simulink model "WSCC_Indian_400kV_Legacy"  (R2022a)
settings: Solver=FixedStepDiscrete  StartTime=0.0  StopTime=1  FixedStep=5e-7  RelTol=1e-3
PreLoadFcn:
  | tf=1e-3
  | to=20e-3
model workspace (MAT data in the model file):
  tf = 0.001
  to = 0.02
undefined symbols (not defined in the file or in its folder): D1, Delta
libraries: spsFourierLib x72, spsPowerPositiveSequenceLib x24, spsThreePhaseVIMeasurementLib x21, spsThreePhaseBreakerLib x12, spsDistributedParametersLineLib x12, spsLoadFlowBusLib x9, spsRMSLib x6, spsThreePhaseParallelRLCLoadLib x6, spsThreePhaseSeriesRLCLoadLib x3, spsThreePhaseSourceLib x3, spsThreePhaseTransformerTwoWindingsLib x3, spsThreePhaseFaultLib x1
(part 1 of 2)
settings Model: ParameterArgumentNames=tf,to  Creator=MARI  LastModifiedBy=Dell
settings SolverCC: AlgebraicLoopSolver=TrustRegion
settings DataIOCC: SignalLogging=off  DSMLogging=off  LoggingIntervals=[0, inf]
settings DebuggingCC: SFMachineParentedDataDiag=warning  ArithmeticOperatorsInVariantConditions=warning
settings SFSimCC: SimUseLocalCustomCode=off  CustomCodeUndefinedFunction=UseInterfaceOnly
settings RTWCC: RTWUseLocalCustomCode=off  DLArmComputeVersion=19.05

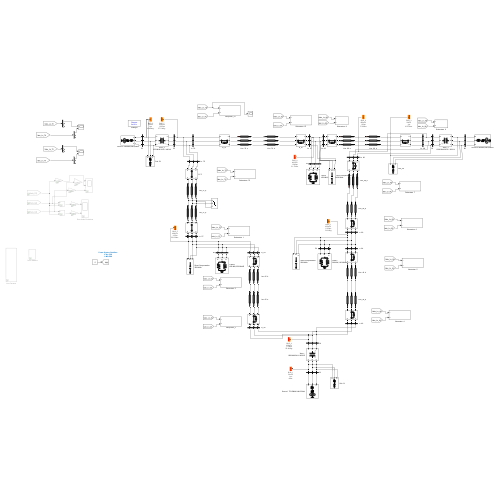
[thumbnail: Simulink's stored preview of the top-level diagram]
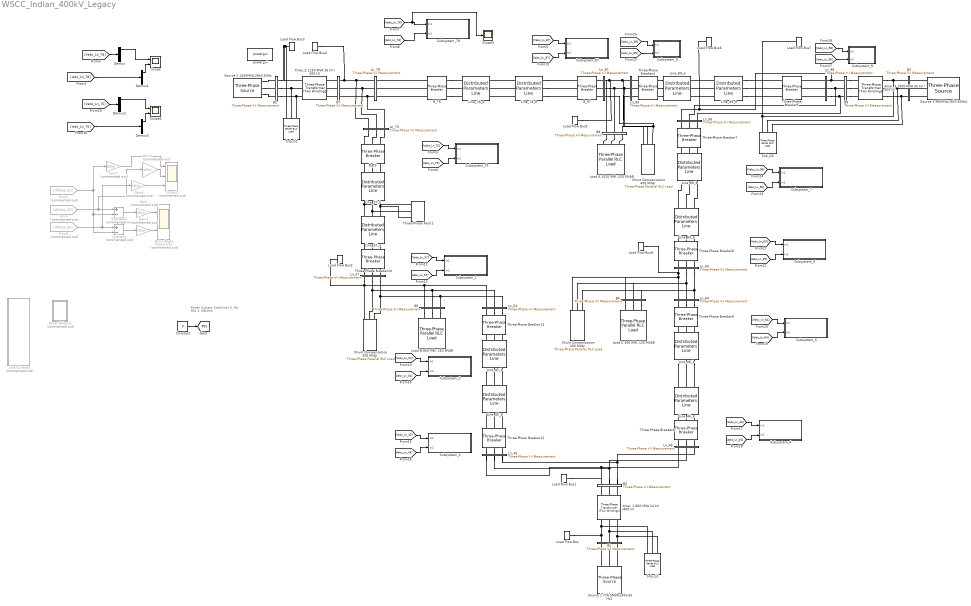
== system WSCC_Indian_400kV_Legacy ==
  note: Power System Stabilizer
      | 0: No PSS
      | 1: MB-PSS
  B1 : spsThreePhaseVIMeasurementLib/Three-Phase V-I Measurement  VoltageMeasurement=phase-to-ground  SetLabelV=on  LabelV=Vabc_G1  Vpu=off  VpuLL=off  CurrentMeasurement=yes  SetLabelI=on  LabelI=Iabc_G1  Ipu=off  Pbase=100e6  Vbase=500e3  OutputType=Complex  PhasorSimulation=off  PSBequivalent=0
  B2 : spsThreePhaseVIMeasurementLib/Three-Phase V-I Measurement  VoltageMeasurement=phase-to-ground  SetLabelV=on  LabelV=Vabc_G2  Vpu=off  VpuLL=off  CurrentMeasurement=yes  SetLabelI=on  LabelI=Iabc_G2  Ipu=off  Pbase=100e6  Vbase=500e3  OutputType=Complex  PhasorSimulation=off  PSBequivalent=0
  B3 : spsThreePhaseVIMeasurementLib/Three-Phase V-I Measurement  VoltageMeasurement=phase-to-ground  SetLabelV=on  LabelV=Vabc_G3  Vpu=off  VpuLL=off  CurrentMeasurement=yes  SetLabelI=on  LabelI=Iabc_G3  Ipu=off  Pbase=100e6  Vbase=500e3  OutputType=Complex  PhasorSimulation=off  PSBequivalent=0
  B4 : spsThreePhaseVIMeasurementLib/Three-Phase V-I Measurement  VoltageMeasurement=phase-to-ground  SetLabelV=on  LabelV=Vabc_X1  Vpu=off  VpuLL=off  CurrentMeasurement=yes  SetLabelI=on  LabelI=Iabc_X1  Ipu=off  Pbase=100e6  Vbase=500e3  OutputType=Complex  PhasorSimulation=off  PSBequivalent=0
  B5 : spsThreePhaseVIMeasurementLib/Three-Phase V-I Measurement  VoltageMeasurement=phase-to-ground  SetLabelV=on  LabelV=Vabc_Ld_B  Vpu=off  VpuLL=off  CurrentMeasurement=yes  SetLabelI=on  LabelI=Iabc_Ld_B  Ipu=off  Pbase=100e6  Vbase=500e3  OutputType=Complex  PhasorSimulation=off  PSBequivalent=0
  B6 : spsThreePhaseVIMeasurementLib/Three-Phase V-I Measurement  VoltageMeasurement=phase-to-ground  SetLabelV=on  LabelV=Vabc_Ld_C  Vpu=off  VpuLL=off  CurrentMeasurement=yes  SetLabelI=on  LabelI=Iabc_Ld_C  Ipu=off  Pbase=100e6  Vbase=500e3  OutputType=Complex  PhasorSimulation=off  PSBequivalent=0
  B7 : spsThreePhaseVIMeasurementLib/Three-Phase V-I Measurement  VoltageMeasurement=phase-to-ground  SetLabelV=on  LabelV=Vabc_X2  Vpu=off  VpuLL=off  CurrentMeasurement=yes  SetLabelI=on  LabelI=Iabc_X2  Ipu=off  Pbase=100e6  Vbase=500e3  OutputType=Complex  PhasorSimulation=off  PSBequivalent=0
  B8 : spsThreePhaseVIMeasurementLib/Three-Phase V-I Measurement  VoltageMeasurement=phase-to-ground  SetLabelV=on  LabelV=Vabc_Ld_A  Vpu=off  VpuLL=off  CurrentMeasurement=yes  SetLabelI=on  LabelI=Iabc_Ld_A  Ipu=off  Pbase=100e6  Vbase=500e3  OutputType=Complex  PhasorSimulation=off  PSBequivalent=0
  B9 : spsThreePhaseVIMeasurementLib/Three-Phase V-I Measurement  VoltageMeasurement=phase-to-ground  SetLabelV=on  LabelV=Vabc_X3  Vpu=off  VpuLL=off  CurrentMeasurement=yes  SetLabelI=on  LabelI=Iabc_X3  Ipu=off  Pbase=100e6  Vbase=500e3  OutputType=Complex  PhasorSimulation=off  PSBequivalent=0
  B_75 : spsThreePhaseBreakerLib/Three-Phase Breaker  InitialState=closed  SwitchA=on  SwitchB=on  SwitchC=on  SwitchTimes=[(0.5+(10/50)) ]  External=off  BreakerResistance=0.01  SnubberResistance=inf  SnubberCapacitance=inf  Measurements=None
  B_78 : spsThreePhaseBreakerLib/Three-Phase Breaker  InitialState=closed  SwitchA=on  SwitchB=on  SwitchC=on  SwitchTimes=[500 501]  External=off  BreakerResistance=0.01  SnubberResistance=10e6  SnubberCapacitance=inf  Measurements=None
  B_87 : spsThreePhaseBreakerLib/Three-Phase Breaker  InitialState=closed  SwitchA=on  SwitchB=on  SwitchC=on  SwitchTimes=[500 501]  External=off  BreakerResistance=0.01  SnubberResistance=10e6  SnubberCapacitance=inf  Measurements=None
  Constant : Constant  Value=0
  Demux{,1..3} (4 alike) : Demux  Outputs=3
  From : From  Commented=on  GotoTag=dtheta_G2
  From1 : From  Commented=on  GotoTag=dtheta_G1
  From2 : From  Commented=on  GotoTag=dtheta_G3
  Gain{,1..4} (5 alike) : Gain  Commented=on  Gain=180/pi
  Line Currents : Subsystem  Commented=on
  Line_45_a : spsDistributedParametersLineLib/Distributed Parameters Line  Phases=3  Length=75  Frequency=50  Resistance=[0.0298 0.1619]  Inductance=[1.0568e-03 3.9470e-03]  Capacitance=[11.0414e-09 7.1301e-09]  x1=[-0.0004 -0.000502991998355344 0 0;-0.00038 -0.000503285101497421 0 0;-0.00036 -0.000503558335805453 0 0;-0.00034 -0.000503811690492617 0 0;-0.00032 -0.000504045155556905 0 0;-0.0003 -0.000504258721781514 0 0;-0.00028 -0.000504452380735217 0 0;-0.00026 -0.000504626124772689 321740.825999906 -262623.935279686;-0.00024 -0.000504779947034814 323384.5791028 -260597.20737983;-0.00022 -0.000504913841448951 325015.565536233 -258560.19154844;-0.0002 -0.000505027802729179 326633.720911655 -256512.968203414;-0.00018 -0.000505121826376501 328238.981347062 -254455.618165624;-0.00016 -0.000505195908679025 329831.283469521 -252388.222655726;-0.00014 -0.000505250046712109 331410.564417669 -250310.863290956;-0.00012 -0.000505284238338474 332976.761844201 -248223.622081904;-0.0001 -0.000505298482208296 334529.813918322 -246126.581429279;-8e-05 -0.000505292777759249 336069.659328196 -244019.824120655;-6e-05 -0.000505267125216536 337596.237283364 -241903.433327204;-4e-05 -0.000505221525592876 339109.487517141 -239777.492600411;-2e-05 -0.000505155980688463 340609.350288999 -237642.085868774]  x2=[-0.0004 -0.000305148640405144 0 0;-0.00038 -0.000306750512833648 0 0;-0.00036 -0.000308340275277147 0 0;-0.00034 -0.000309917864974541 0 0;-0.00032 -0.00031148321964529 0 0;-0.0003 -0.000313036277491872 0 0;-0.00028 -0.000314576977202222 0 0;-0.00026 -0.000316105257952155 311271.717606713 -279950.706951068;-0.00024 -0.000317621059407763 313024.543961436 -277989.415950935;-0.00022 -0.0003191243217278 314765.012643147 -276017.150404654;-0.0002 -0.000320614985566043 316493.054941124 -274033.988173893;-0.00018 -0.000322092992073637 318208.602635214 -272040.0075505;-0.00016 -0.000323558282901415 319911.587998532 -270035.287253415;-0.00014 -0.000325010800202205 321601.943800133 -268019.906425565;-0.00012 -0.00032645048663311 323279.603307663 -265993.944630732;-0.0001 -0.000327877285357777 324944.500289998 -263957.48185042;-8e-05 -0.000329291140048632 326596.569019855 -261910.598480692;-6e-05 -0.000330691994889116 328235.744276391 -259853.375328999;-4e-05 -0.000332079794575877 329861.961347772 -257785.893610988;-2e-05 -0.000333454484320959 331475.156033733 -255708.234947298]  x3=[-0.0004 1.79056945115255e-06 0 0;-0.00038 1.80115317620371e-06 0 0;-0.00036 1.81166579481155e-06 0 0;-0.00034 1.82210689195587e-06 0 0;-0.00032 1.83247605544005e-06 0 0;-0.0003 1.84277287590726e-06 0 0;-0.00028 1.85299694685666e-06 0 0;-0.00026 1.86314786465944e-06 274.455148622571 -531.709356408434;-0.00024 1.87322522857474e-06 277.790537542582 -529.974419725581;-0.00022 1.88322864076549e-06 281.114959767823 -528.218560560099;-0.0002 1.89315770631411e-06 284.428284055799 -526.441848230301;-0.00018 1.90301203323809e-06 287.73037960214 -524.644352877748;-0.00016 1.91279123250548e-06 291.021116045767 -522.826145464478;-0.00014 1.92249491805023e-06 294.300363474041 -520.987297770207;-0.00012 1.93212270678745e-06 297.567992427888 -519.127882389493;-0.0001 1.94167421862854e-06 300.823873906911 -517.247972728872;-8e-05 1.95114907649615e-06 304.067879374486 -515.347643003957;-6e-05 1.96054690633912e-06 307.299880762831 -513.426968236514;-4e-05 1.96986733714723e-06 310.519750478065 -511.486024251492;-2e-05 1.97911000096581e-06 313.727361405245 -509.524887674037]  x4=[-0.0004 -2.83815574986041e-06 0 0;-0.00038 -2.85167951589665e-06 0 0;-0.00036 -2.86509070250846e-06 0 0;-0.00034 -2.87838878024516e-06 0 0;-0.00032 -2.89157322412141e-06 0 0;-0.0003 -2.90464351363793e-06 0 0;-0.00028 -2.91759913280208e-06 0 0;-0.00026 -2.9304395701482e-06 1690.23052973685 -1294.68064107459;-0.00024 -2.94316431875781e-06 1698.33183087633 -1284.03512342686;-0.00022 -2.95577287627961e-06 1706.36608478314 -1273.33891427108;-0.0002 -2.96826474494935e-06 1714.33297427868 -1262.59243587526;-0.00018 -2.98063943160945e-06 1722.23218484381 -1251.79611249199;-0.00016 -2.99289644772846e-06 1730.06340463121 -1240.95037034161;-0.00014 -3.00503530942037e-06 1737.82632447774 -1230.05563759546;-0.00012 -3.01705553746371e-06 1745.52063791662 -1219.11234435892;-0.0001 -3.02895665732046e-06 1753.14604118952 -1208.12092265449;-8e-05 -3.04073819915478e-06 1760.70223325858 -1197.08180640467;-6e-05 -3.05239969785157e-06 1768.18891581828 -1185.99543141486;-4e-05 -3.06394069303484e-06 1775.60579330721 -1174.86223535616;-2e-05 -3.07536072908586e-06 1782.95257291974 -1163.68265774811]  x5=0.000397871322084792  V1=[1.62e-10 4.153e+05 4.153e+05;314.2 314.2 314.2;-0.6943 0.8874 -0.6834]  V2=[8.471e-10 4.186e+05 4.186e+05;314.2 314.2 314.2;-0.039 0.8395 -0.7313]  I1=[7.601e-12 598 598;314.2 314.2 314.2;-1.312 0.4775 -1.093]  I2=[4.421e-12 2129 2129;314.2 314.2 314.2;2.105 0.9183 -0.6525]  nHarmo=1  Measurements=None  Decoupling=off  VsMag0=0  VrMag0=0  VsAngle0=0  VrAngle0=0  IsMag0=0  IrMag0=0  IsAngle0=0  IrAngle0=0
      settings: SourceProductBaseCode=PS
  Line_45_b : spsDistributedParametersLineLib/Distributed Parameters Line  Phases=3  Length=75  Frequency=50  Resistance=[0.0298 0.1619]  Inductance=[1.0568e-03 3.9470e-03]  Capacitance=[11.0414e-09 7.1301e-09]  x1=[-0.0004 -0.000305148627791813 0 0;-0.00038 -0.000306750500118396 0 0;-0.00036 -0.000308340262460476 0 0;-0.00034 -0.000309917852056956 0 0;-0.00032 -0.000311483206627302 0 0;-0.0003 -0.000313036264373994 0 0;-0.00028 -0.000314576963984974 0 0;-0.00026 -0.000316105244636057 311271.717606713 -279950.706951068;-0.00024 -0.00031762104599334 313024.543961436 -277989.415950935;-0.00022 -0.000319124308215583 314765.012643147 -276017.150404654;-0.0002 -0.000320614971956565 316493.054941124 -274033.988173893;-0.00018 -0.000322092978367435 318208.602635214 -272040.0075505;-0.00016 -0.00032355826909903 319911.587998532 -270035.287253415;-0.00014 -0.000325010786304183 321601.943800133 -268019.906425565;-0.00012 -0.000326450472639999 323279.603307663 -265993.944630732;-0.0001 -0.000327877271270129 324944.500289998 -263957.48185042;-8e-05 -0.000329291125867004 326596.569019855 -261910.598480692;-6e-05 -0.000330691980614067 328235.744276391 -259853.375328999;-4e-05 -0.000332079780207971 329861.961347772 -257785.893610988;-2e-05 -0.000333454469860763 331475.156033733 -255708.234947298]  x2=[-0.0004 -0.000103064623526066 0 0;-0.00038 -0.000105946361861863 0 0;-0.00036 -0.000108823917616703 0 0;-0.00034 -0.000111697177189612 0 0;-0.00032 -0.000114566027149221 0 0;-0.0003 -0.000117430354238247 0 0;-0.00028 -0.000120290045377961 0 0;-0.00026 -0.000123144987672653 298949.882553439 -295284.144230629;-0.00024 -0.000125995068414089 300799.294324294 -293399.970425258;-0.00022 -0.000128840175085963 302636.83105406 -291504.213691436;-0.0002 -0.000131680195368334 304462.420199933 -289596.948870392;-0.00018 -0.000134515017142064 306275.989690779 -287678.251257676;-0.00016 -0.000137344528493244 308077.467929982 -285748.196600185;-0.00014 -0.000140168617717611 309866.783798263 -283806.861093171;-0.00012 -0.000142987173324957 311643.866656497 -281854.321377236;-0.0001 -0.000145800084043534 313408.646348495 -279890.654535305;-8e-05 -0.000148607238824443 315161.053203777 -277915.938089583;-6e-05 -0.000151408526846019 316901.018040321 -275930.249998493;-4e-05 -0.000154203837518208 318628.472167293 -273933.668653602;-2e-05 -0.000156993060486931 320343.347387764 -271926.272876522]  x3=[-0.0004 2.02786013516334e-06 0 0;-0.00038 2.03713024797852e-06 0 0;-0.00036 2.04631993837963e-06 0 0;-0.00034 2.05542884357343e-06 0 0;-0.00032 2.06445660395595e-06 0 0;-0.0003 2.07340286312666e-06 0 0;-0.00028 2.08226726790257e-06 0 0;-0.00026 2.09104946833215e-06 311.165075108754 -505.329069968942;-0.00024 2.09974911770918e-06 314.333988267489 -503.364000256953;-0.00022 2.10836587258638e-06 317.490492058594 -501.37905859613;-0.0002 2.11689939278903e-06 320.634461868702 -499.374323348573;-0.00018 2.12534934142837e-06 323.765773579271 -497.349873657795;-0.00016 2.13371538491489e-06 326.884303571474 -495.305789445605;-0.00014 2.14199719297152e-06 329.989928731088 -493.242151408947;-0.00012 2.15019443864666e-06 333.082526453349 -491.159041016718;-0.0001 2.15830679832708e-06 336.161974647794 -489.056540506547;-8e-05 2.16633395175072e-06 339.228151743082 -486.934732881557;-6e-05 2.1742755820193e-06 342.28093669179 -484.793701907078;-4e-05 2.18213137561086e-06 345.320208975196 -482.633532107348;-2e-05 2.18990102239212e-06 348.345848608036 -480.454308762171]  x4=[-0.0004 -2.51020404096927e-06 0 0;-0.00038 -2.52564213893374e-06 0 0;-0.00036 -2.54098052887116e-06 0 0;-0.00034 -2.55621860524815e-06 0 0;-0.00032 -2.57135576649156e-06 0 0;-0.0003 -2.58639141501217e-06 0 0;-0.00028 -2.60132495722833e-06 0 0;-0.00026 -2.61615580358936e-06 1576.01556289566 -1423.10339701304;-0.00024 -2.63088336859883e-06 1584.92601720433 -1413.17297349099;-0.00022 -2.64550707083772e-06 1593.77390134767 -1403.18676031967;-0.0002 -2.66002633298727e-06 1602.55886602637 -1393.14515173771;-0.00018 -2.6744405818519e-06 1611.28056442505 -1383.0485441706;-0.00016 -2.68874924838173e-06 1619.93865222601 -1372.89733621512;-0.00014 -2.70295176769511e-06 1628.53278762276 -1362.69192862359;-0.00012 -2.71704757910089e-06 1637.06263133354 -1352.43272428801;-0.0001 -2.73103612612059e-06 1645.52784661474 -1342.12012822422;-8e-05 -2.7449168565103e-06 1653.92809927415 -1331.75454755584;-6e-05 -2.75868922228258e-06 1662.26305768418 -1321.33639149826;-4e-05 -2.77235267972799e-06 1670.53239279494 -1310.86607134243;-2e-05 -2.78590668943663e-06 1678.73577814725 -1300.34400043866]  x5=0.000397871322084792  V1=[8.377e-10 4.186e+05 4.186e+05;314.2 314.2 314.2;-0.02057 0.8395 -0.7313]  V2=[8.866e-10 4.202e+05 4.202e+05;314.2 314.2 314.2;-0.5299 0.7927 -0.7781]  I1=[5.663e-12 593.1 593.1;314.2 314.2 314.2;-2.774 0.5529 -1.018]  I2=[8.582e-12 2124 2124;314.2 314.2 314.2;-0.07241 0.8375 -0.7333]  nHarmo=1  Measurements=None  Decoupling=off  VsMag0=0  VrMag0=0  VsAngle0=0  VrAngle0=0  IsMag0=0  IrMag0=0  IsAngle0=0  IrAngle0=0
      settings: SourceProductBaseCode=PS
  Line_46_a : spsDistributedParametersLineLib/Distributed Parameters Line  Phases=3  Length=90  Frequency=50  Resistance=[0.0298 0.1619]  Inductance=[1.0568e-03 3.9470e-03]  Capacitance=[11.0414e-09 7.1301e-09]  x1=[-0.00048 -0.000501780155719701 302839.15593119 -284220.468288801;-0.00046 -0.000502153472113537 304618.976263006 -282312.076006295;-0.00044 -0.000502506964348118 306386.77075923 -280392.538526423;-0.00042 -0.000502840618468176 308142.469630363 -278461.931629239;-0.0004 -0.000503154421301618 309886.003564419 -276520.331531798;-0.00038 -0.000503448360460045 311617.303729664 -274567.814885147;-0.00036 -0.000503722424339243 313336.301777333 -272604.458771299;-0.00034 -0.000503976602119639 315042.929844324 -270630.340700193;-0.00032 -0.00050421088376673 316737.120555886 -268645.538606629;-0.0003 -0.000504425260031477 318418.807028269 -266650.130847196;-0.00028 -0.000504619722450672 320087.92287137 -264644.196197175;-0.00026 -0.000504794263347272 321744.402191355 -262627.813847432;-0.00024 -0.000504948875830701 323388.179593256 -260601.063401288;-0.00022 -0.000505083553797124 325019.190183556 -258564.024871383;-0.0002 -0.000505198291929684 326637.36957275 -256516.778676508;-0.00018 -0.000505293085698717 328242.653877885 -254459.405638437;-0.00016 -0.000505367931361927 329834.979725087 -252391.986978737;-0.00014 -0.000505422825964535 331414.284252057 -250314.604315555;-0.00012 -0.000505457767339397 332980.505110557 -248227.339660401;-0.0001 -0.000505472754107086 334533.58046887 -246130.275414912;-8e-05 -0.000505467785675951 336073.449014239 -244023.494367591;-6e-05 -0.000505442862242137 337600.04995529 -241907.079690548;-4e-05 -0.000505397984789579 339113.323024433 -239781.11493621;-2e-05 -0.000505333155089961 340613.208480238 -237645.684034025]  x2=[-0.00048 -0.000411589322638186 301824.904517896 -295099.84373655;-0.00046 -0.000412724558984348 303673.101552408 -293197.609392173;-0.00044 -0.000413843501671618 305509.310092842 -291283.800108212;-0.00042 -0.000414946106526057 307333.45764883 -289358.491438581;-0.0004 -0.000416032330018711 309145.472206149 -287421.759391168;-0.00038 -0.000417102129267337 310945.282229567 -285473.68042484;-0.00036 -0.000418155462038093 312732.816665666 -283514.331446418;-0.00034 -0.000419192286747205 314508.004945647 -281543.789807644;-0.00032 -0.000420212562462608 316270.776988118 -279562.13330213;-0.0003 -0.000421216248905564 318021.063201855 -277569.440162279;-0.00028 -0.000422203306452252 319758.794488556 -275565.789056206;-0.00026 -0.000423173696135328 321483.902245565 -273551.259084625;-0.00024 -0.00042412737964547 323196.318368583 -271525.92977773;-0.00022 -0.000425064319332886 324895.975254352 -269489.881092055;-0.0002 -0.000425984478208802 326582.805803329 -267443.193407314;-0.00018 -0.000426887819946921 328256.743422332 -265385.947523234;-0.00016 -0.000427774308884856 329917.72202717 -263318.22465636;-0.00014 -0.000428643910025544 331565.676045253 -261240.106436848;-0.00012 -0.00042949658903862 333200.540418176 -259151.67490525;-0.0001 -0.000430332312261777 334822.250604295 -257053.012509265;-8e-05 -0.000431151046702093 336430.742581267 -254944.202100491;-6e-05 -0.000431952760037334 338025.952848584 -252825.326931153;-4e-05 -0.00043273742061723 339607.818430075 -250696.470650814;-2e-05 -0.000433504997464725 341176.276876397 -248557.717303074]  x3=[-0.00048 5.03743589015423e-07 565.121573651507 -958.528765308815;-0.00046 5.07008815739957e-07 571.132992855913 -954.959104569544;-0.00044 5.10254026624583e-07 577.121864707697 -951.351743679977;-0.00042 5.13479093553934e-07 583.087952776453 -947.706825052544;-0.0004 5.16683889207888e-07 589.031021531241 -944.024492582392;-0.00038 5.198682870666e-07 594.950836349881 -940.304891641702;-0.00036 5.23032161415496e-07 600.84716352822 -936.54816907395;-0.00034 5.26175387350234e-07 606.719770289359 -932.75447318811;-0.00032 5.29297840781636e-07 612.568424792837 -928.9239537528;-0.0003 5.32399398440587e-07 618.39289614379 -925.056761990368;-0.00028 5.35479937882902e-07 624.192954402061 -921.153050570924;-0.00026 5.38539337494157e-07 629.968370591282 -917.21297360631;-0.00024 5.41577476494495e-07 635.718916707911 -913.236686644018;-0.00022 5.4459423494339e-07 641.444365730233 -909.224346661049;-0.0002 5.47589493744385e-07 647.144491627325 -905.176112057716;-0.00018 5.50563134649789e-07 652.819069367976 -901.092142651388;-0.00016 5.53515040265353e-07 658.467874929574 -896.972599670185;-0.00014 5.56445094054897e-07 664.090685306947 -892.817645746611;-0.00012 5.59353180344914e-07 669.687278521169 -888.627444911131;-0.0001 5.62239184329137e-07 675.257433628324 -884.402162585699;-8e-05 5.6510299207307e-07 680.800930728226 -880.141965577228;-6e-05 5.67944490518488e-07 686.317550973099 -875.847022071;-4e-05 5.70763567487897e-07 691.807076576225 -871.517501624032;-2e-05 5.73560111688965e-07 697.269290820531 -867.153575158376]  x4=[-0.00048 -1.68914033558431e-06 1286.57292882659 -995.934322856657;-0.00046 -1.694977924365e-06 1292.80513169933 -987.830941038064;-0.00044 -1.70074859831951e-06 1298.98629683911 -979.688561345357;-0.00042 -1.7064521296315e-06 1305.11618022411 -971.507505225743;-0.0004 -1.71208829313533e-06 1311.19453985704 -963.28809565331;-0.00038 -1.71765686632491e-06 1317.22113577465 -955.030657116274;-0.00036 -1.7231576293625e-06 1323.19573005727 -946.735515604169;-0.00034 -1.72859036508741e-06 1329.11808683814 -938.40299859498;-0.00032 -1.73395485902453e-06 1334.98797231275 -930.033435042209;-0.0003 -1.73925089939281e-06 1340.80515474808 -921.627155361894;-0.00028 -1.74447827711367e-06 1346.56940449173 -913.184491419565;-0.00026 -1.74963678581917e-06 1352.28049398099 -904.705776517137;-0.00024 -1.75472622186022e-06 1357.93819775182 -896.191345379756;-0.00022 -1.7597463843146e-06 1363.54229244776 -887.641534142585;-0.0002 -1.7646970749949e-06 1369.09255682876 -879.056680337532;-0.00018 -1.76957809845633e-06 1374.58877177988 -870.437122879925;-0.00016 -1.77438926200443e-06 1380.03072031996 -861.783202055134;-0.00014 -1.77913037570271e-06 1385.41818761019 -853.095259505135;-0.00012 -1.78380125238012e-06 1390.75096096259 -844.373638215024;-0.0001 -1.78840170763844e-06 1396.0288298484 -835.618682499475;-8e-05 -1.79293155985957e-06 1401.25158590639 -826.83073798915;-6e-05 -1.79739063021271e-06 1406.41902295109 -818.01015161705;-4e-05 -1.8017787426614e-06 1411.53093698095 -809.157271604822;-2e-05 -1.80609572397047e-06 1416.58712618634 -800.272447449009]  x5=0.00047744558650175  V1=[2.78e-10 4.153e+05 4.153e+05;314.2 314.2 314.2;2.169 0.8713 -0.6995]  V2=[5.247e-10 4.221e+05 4.221e+05;314.2 314.2 314.2;2.009 0.8508 -0.72]  I1=[2.389e-12 1113 1113;314.2 314.2 314.2;0.1121 0.5869 -0.9839]  I2=[3.387e-12 1627 1627;314.2 314.2 314.2;-2.917 0.9662 -0.6046]  nHarmo=1  Measurements=None  Decoupling=off  VsMag0=0  VrMag0=0  VsAngle0=0  VrAngle0=0  IsMag0=0  IrMag0=0  IsAngle0=0  IrAngle0=0
      settings: SourceProductBaseCode=PS
  Line_46_b : spsDistributedParametersLineLib/Distributed Parameters Line  Phases=3  Length=30  Frequency=50  Resistance=[0.0298 0.1619]  Inductance=[1.0568e-03 3.9470e-03]  Capacitance=[11.0414e-09 7.1301e-09]  x1=[-0.00016 -0.000427774308702069 0 0;-0.00014 -0.000428643909865589 0 0;-0.00012 -0.000429496588901504 333200.540418176 -259151.67490525;-0.0001 -0.000430332312147506 334822.250604295 -257053.012509265;-8e-05 -0.00043115104661067 336430.742581267 -254944.202100491;-6e-05 -0.000431952759968763 338025.952848584 -252825.326931153;-4e-05 -0.000432737420571515 339607.818430075 -250696.470650814;-2e-05 -0.000433504997441867 341176.276876397 -248557.717303074]  x2=[-0.00016 -0.000399750126995155 0 0;-0.00014 -0.000400886003436956 0 0;-0.00012 -0.000402006053585768 332630.691588008 -262198.669447582;-0.0001 -0.000403110233223929 334271.557727847 -260103.527348785;-8e-05 -0.000404198498760318 335899.227398951 -257998.116808096;-6e-05 -0.000405270807232074 337513.636343708 -255882.520943518;-4e-05 -0.000406327116306296 339114.720828019 -253756.823275156;-2e-05 -0.00040736738428171 340702.417643809 -251621.107721911]  x3=[-0.00016 6.4357650210188e-07 0 0;-0.00014 6.4602632630302e-07 0 0;-0.00012 6.48450646490972e-07 753.040289841409 -823.678614845093;-0.0001 6.50849366957726e-07 758.200716781565 -818.930895583143;-8e-05 6.53222393005905e-07 763.33121125567 -814.150846331669;-6e-05 6.55569630952504e-07 768.431570720586 -809.338655798831;-4e-05 6.57890988132588e-07 773.501593822857 -804.494513961673;-2e-05 6.6018637290295e-07 778.54108040665 -799.618612058618]  x4=[-0.00016 -1.7395987457411e-06 0 0;-0.00014 -1.74490522315752e-06 0 0;-0.00012 -1.75014281470349e-06 1367.39693584155 -892.4465672657;-0.0001 -1.75531131360786e-06 1372.97731485002 -883.837399334052;-8e-05 -1.76041051582714e-06 1378.50349106502 -875.193339015251;-6e-05 -1.76544022005356e-06 1383.97524632256 -866.514727561996;-4e-05 -1.77040022772301e-06 1389.39236460713 -857.801907591008;-2e-05 -1.77529034302289e-06 1394.75463206016 -849.0552230695]  x5=0.000159148528833917  V1=[5.267e-10 4.221e+05 4.221e+05;314.2 314.2 314.2;2.115 0.9152 -0.6556]  V2=[4.511e-10 4.235e+05 4.235e+05;314.2 314.2 314.2;1.521 0.9087 -0.6621]  I1=[7.622e-12 1116 1116;314.2 314.2 314.2;-1.047 0.7461 -0.8247]  I2=[9.859e-12 1633 1633;314.2 314.2 314.2;1.521 0.998 -0.5728]  nHarmo=1  Measurements=None  Decoupling=off  VsMag0=0  VrMag0=0  VsAngle0=0  VrAngle0=0  IsMag0=0  IrMag0=0  IsAngle0=0  IrAngle0=0
      settings: SourceProductBaseCode=PS
  Line_57_a : spsDistributedParametersLineLib/Distributed Parameters Line  Phases=3  Length=30  Frequency=50  Resistance=[0.0298 0.1619]  Inductance=[1.0568e-03 3.9470e-03]  Capacitance=[11.0414e-09 7.1301e-09]  x1=[-0.00016 -0.000137305305694705 0 0;-0.00014 -0.00014012931010315 0 0;-0.00012 -0.000142947782446373 311649.17374747 -281855.555955426;-0.0001 -0.00014576061145591 313413.961091743 -279891.85574391;-8e-05 -0.000148567686086089 315166.375389483 -277917.10588118;-6e-05 -0.00015136889551841 316906.347458374 -275931.38432698;-4e-05 -0.000154164129165921 318633.808607298 -273934.769474197;-2e-05 -0.000156953276677584 320348.690639046 -271927.340145767]  x2=[-0.00016 -0.000142819253464008 0 0;-0.00014 -0.000145971796518761 0 0;-0.00012 -0.000149118576856932 318234.770516593 -270572.457865407;-0.0001 -0.000152259470249021 319928.534537009 -268567.602119856;-8e-05 -0.000155394352697934 321609.668326686 -266552.143785234;-6e-05 -0.00015852310044388 323278.105517342 -264526.162428386;-4e-05 -0.000161645589969256 324933.780241933 -262489.738031587;-2e-05 -0.000164761698003521 326576.627137255 -260442.950989384]  x3=[-0.00016 1.19106734480895e-06 0 0;-0.00014 1.18519076420232e-06 0 0;-0.00012 1.17926739429368e-06 2171.66168617045 -1479.63388710976;-0.0001 1.17329746892755e-06 2180.91557213176 -1465.95981740172;-8e-05 1.16728122378635e-06 2190.08335928061 -1452.22787411021;-6e-05 1.16121889638114e-06 2199.16468568846 -1438.43859934884;-4e-05 1.15511072604223e-06 2208.15919284009 -1424.59253749457;-2e-05 1.14895695390972e-06 2217.06652564776 -1410.69023516622]  x4=[-0.00016 -1.53383949725334e-06 0 0;-0.00014 -1.53601602750111e-06 0 0;-0.00012 -1.53813191846619e-06 -168.781227025331 -334.859258343707;-0.0001 -1.54018708661683e-06 -166.673926497094 -335.913125247926;-8e-05 -1.54218145081851e-06 -164.56004596763 -336.953730877135;-6e-05 -1.54411493233716e-06 -162.439668889323 -337.981034150007;-4e-05 -1.54598745484222e-06 -160.31287897103 -338.994994510367;-2e-05 -1.54779894440972e-06 -158.179760174774 -339.995571928796]  x5=0.000159148528833917  V1=[8.847e-10 4.202e+05 4.202e+05;314.2 314.2 314.2;0.04885 0.841 -0.7298]  V2=[4.139e-10 4.177e+05 4.177e+05;314.2 314.2 314.2;-0.2267 0.8716 -0.6992]  I1=[1.496e-11 2628 2628;314.2 314.2 314.2;1.536 0.9781 -0.5927]  I2=[1.402e-11 375 375;314.2 314.2 314.2;-1.159 -0.4607 -2.031]  nHarmo=1  Measurements=None  Decoupling=off  VsMag0=0  VrMag0=0  VsAngle0=0  VrAngle0=0  IsMag0=0  IrMag0=0  IsAngle0=0  IrAngle0=0
      settings: SourceProductBaseCode=PS
  Line_57_b : spsDistributedParametersLineLib/Distributed Parameters Line  Phases=3  Length=90  Frequency=50  Resistance=[0.0298 0.1619]  Inductance=[1.0568e-03 3.9470e-03]  Capacitance=[11.0414e-09 7.1301e-09]  x1=[-0.00048 -9.16970319348276e-05 285665.838008779 -304758.680171657;-0.00046 -9.49247126624822e-05 287575.041868576 -302957.78491149;-0.00044 -9.8148645925018e-05 289472.892758129 -301144.929396722;-0.00042 -0.00010136870444707 291359.315753532 -299320.185195783;-0.0004 -0.000104584761106242 293234.236382036 -297483.624346452;-0.00038 -0.000107796688938123 295097.580624985 -295635.319353005;-0.00036 -0.000111004361141302 296949.274920739 -293775.343183358;-0.00034 -0.000114207651082373 298789.246167578 -291903.769266187;-0.00032 -0.000117406432300934 300617.421726588 -290020.671488024;-0.0003 -0.00012060057851458 302433.729424527 -288126.124190346;-0.00028 -0.000123789963623888 304238.097556678 -286220.202166635;-0.00026 -0.000126974461717394 306030.454889676 -284302.980659431;-0.00024 -0.000130153947076566 307810.730664324 -282374.535357355;-0.00022 -0.000133328294180767 309578.854598381 -280434.942392125;-0.0002 -0.000136497377712209 311334.756889342 -278484.278335552;-0.00018 -0.000139661072560899 313078.368217192 -276522.620196511;-0.00016 -0.000142819253829583 314809.619747141 -274550.045417908;-0.00014 -0.000145971796838672 316528.443132343 -272566.631873616;-0.00012 -0.000149118577131164 318234.770516593 -270572.457865407;-0.0001 -0.000152259470477564 319928.534537009 -268567.602119856;-8e-05 -0.000155394352880779 321609.668326686 -266552.143785234;-6e-05 -0.00015852310058102 323278.105517342 -264526.162428386;-4e-05 -0.000161645590060686 324933.780241933 -262489.738031587;-2e-05 -0.000164761698049237 326576.627137255 -260442.950989384]  x2=[-0.00048 -9.21193518598346e-05 307474.163519976 -271342.512180013;-0.00046 -9.62856591401417e-05 309172.978307394 -269405.251677202;-0.00044 -0.000100448165227493 310859.587475018 -267457.355516351;-0.00042 -0.000104606705793277 312533.924438405 -265498.900597064;-0.0004 -0.000108761116665431 314195.923097598 -263529.964235789;-0.00038 -0.000112911233834927 315845.517839738 -261550.624162761;-0.00036 -0.000117056893462248 317482.643541647 -259560.958518937;-0.00034 -0.000121197931883847 319107.235572407 -257561.045852911;-0.00032 -0.00012533418561862 320719.229795905 -255550.96511781;-0.0003 -0.000129465491374351 322318.562573371 -253530.795668179;-0.00028 -0.000133591686054164 323905.170765883 -251500.617256849;-0.00026 -0.000137712606762956 325478.991736869 -249460.510031788;-0.00024 -0.000141828090813835 327039.96335457 -247410.554532936;-0.00022 -0.000145937975734538 328588.023994499 -245350.831689026;-0.0002 -0.000150042099273844 330123.112541875 -243281.422814388;-0.00018 -0.000154140299407984 331645.168394028 -241202.409605743;-0.00016 -0.000158232414347034 333154.131462801 -239113.87413897;-0.00014 -0.000162318282541303 334649.942176914 -237015.898865876;-0.00012 -0.000166397742687711 336132.541484324 -234908.56661093;-0.0001 -0.000170470633736155 337601.870854546 -232791.960568002;-8e-05 -0.000174536794895873 339057.872280974 -230666.164297075;-6e-05 -0.000178596065641783 340500.488283165 -228531.261720945;-4e-05 -0.000182648285720826 341929.661909108 -226387.337121911;-2e-05 -0.000186693295158294 343345.336737476 -224234.475138444]  x3=[-0.00048 1.23785488124962e-06 2040.99402128711 -1646.0438750609;-0.00046 1.2324041301442e-06 2051.29606442935 -1633.18752431424;-0.00044 1.22690472583395e-06 2061.51712591535 -1620.26669812058;-0.00042 1.22135688542591e-06 2071.65680223509 -1607.28190657202;-0.0004 1.21576082793934e-06 2081.71469309153 -1594.23366228589;-0.00038 1.21011677429699e-06 2091.69040141636 -1581.12248038455;-0.00036 1.20442494731645e-06 2101.58353338568 -1567.94887847499;-0.00034 1.19868557170129e-06 2111.39369843559 -1554.71337662847;-0.00032 1.19289887403224e-06 2121.12050927757 -1541.41649735993;-0.0003 1.18706508275822e-06 2130.76358191379 -1528.05876560741;-0.00028 1.18118442818731e-06 2140.32253565225 -1514.64070871128;-0.00026 1.17525714247768e-06 2149.79699312181 -1501.16285639345;-0.00024 1.16928345962843e-06 2159.18658028713 -1487.62574073645;-0.00022 1.16326361547033e-06 2168.49092646338 -1474.02989616243;-0.0002 1.15719784765652e-06 2177.7096643309 -1460.37585941205;-0.00018 1.15108639565312e-06 2186.84242994972 -1446.66416952331;-0.00016 1.1449295007298e-06 2195.88886277387 -1432.89536781024;-0.00014 1.13872740595022e-06 2204.84860566568 -1419.06999784155;-0.00012 1.13248035616247e-06 2213.72130490985 -1405.18860541919;-0.0001 1.12618859798938e-06 2222.5066102274 -1391.25173855676;-8e-05 1.11985237981878e-06 2231.20417478951 -1377.25994745789;-6e-05 1.11347195179372e-06 2239.81365523124 -1363.21378449455;-4e-05 1.10704756580257e-06 2248.33471166504 -1349.11380418519;-2e-05 1.10057947546909e-06 2256.76700769418 -1334.96056317289]  x4=[-0.00048 -1.36356553672137e-06 -225.806870609764 -296.28896755923;-0.00046 -1.36802539695598e-06 -223.940787135922 -297.701896136061;-0.00044 -1.37243124989035e-06 -222.065862863252 -299.10307195178;-0.00042 -1.37678292158896e-06 -220.182171810554 -300.492439690365;-0.0004 -1.38108024025525e-06 -218.289788342725 -301.869944501957;-0.00038 -1.38532303623845e-06 -216.388787167824 -303.235532005023;-0.00036 -1.38951114204023e-06 -214.479243334123 -304.589148288509;-0.00034 -1.39364439232134e-06 -212.561232227142 -305.93073991396;-0.00032 -1.39772262390815e-06 -210.634829566676 -307.260253917637;-0.0003 -1.40174567579905e-06 -208.700111403803 -308.577637812603;-0.00028 -1.40571338917084e-06 -206.757154117884 -309.882839590798;-0.00026 -1.409625607385e-06 -204.806034413545 -311.17580772509;-0.00024 -1.41348217599384e-06 -202.846829317652 -312.456491171311;-0.00022 -1.41728294274664e-06 -200.879616176267 -313.724839370272;-0.0002 -1.42102775759564e-06 -198.904472651596 -314.980802249758;-0.00018 -1.42471647270196e-06 -196.921476718923 -316.224330226504;-0.00016 -1.42834894244144e-06 -194.930706663534 -317.455374208156;-0.00014 -1.4319250234104e-06 -192.93224107762 -318.673885595205;-0.00012 -1.43544457443128e-06 -190.926158857181 -319.879816282907;-0.0001 -1.43890745655824e-06 -188.912539198909 -321.073118663185;-8e-05 -1.44231353308262e-06 -186.891461597059 -322.253745626503;-6e-05 -1.44566266953835e-06 -184.863005840315 -323.421650563731;-4e-05 -1.44895473370726e-06 -182.827252008636 -324.576787367981;-2e-05 -1.45218959562428e-06 -180.784280470098 -325.71911043643]  x5=0.00047744558650175  V1=[4.309e-10 4.177e+05 4.177e+05;314.2 314.2 314.2;-0.354 0.8072 -0.7636]  V2=[3.73e-10 4.101e+05 4.101e+05;314.2 314.2 314.2;-0.5088 0.9019 -0.6689]  I1=[1.704e-12 2622 2622;314.2 314.2 314.2;-1.588 0.9462 -0.6246]  I2=[3.147e-12 372.5 372.5;314.2 314.2 314.2;-0.7702 -0.5974 -2.168]  nHarmo=1  Measurements=None  Decoupling=off  VsMag0=0  VrMag0=0  VsAngle0=0  VrAngle0=0  IsMag0=0  IrMag0=0  IsAngle0=0  IrAngle0=0
      settings: SourceProductBaseCode=PS
  Line_69_a : spsDistributedParametersLineLib/Distributed Parameters Line  Phases=3  Length=70  Frequency=50  Resistance=[0.0298 0.1619]  Inductance=[1.0568e-03 3.9470e-03]  Capacitance=[11.0414e-09 7.1301e-09]  x1=[-0.00038 -0.000386210445846985 310131.617493116 -288465.740037434;-0.00036 -0.000387517233677351 311937.967531581 -286511.444371006;-0.00034 -0.000388808722990867 313732.002793211 -284545.837723341;-0.00032 -0.000390084862801746 315513.652452566 -282568.997693223;-0.0003 -0.000391345602730174 317282.846173168 -280581.002322911;-0.00028 -0.000392590893004298 319039.514110279 -278581.930095059;-0.00026 -0.000393820684462189 320783.586913655 -276571.859929616;-0.00024 -0.000395034928553786 322514.99573029 -274550.87118071;-0.00022 -0.000396233577342812 324233.672207128 -272519.043633515;-0.0002 -0.000397416583508665 325939.548493763 -270476.457501106;-0.00018 -0.000398583900348288 327632.557245122 -268423.193421284;-0.00016 -0.000399735481778009 329312.631624118 -266359.3324534;-0.00014 -0.000400871282335367 330979.705304291 -264284.956075151;-0.00012 -0.0004019912571809 332633.712472426 -262200.146179365;-0.0001 -0.000403095362099919 334274.587831153 -260104.985070766;-8e-05 -0.000404183553504251 335902.266601523 -257999.555462727;-6e-05 -0.000405255788433965 337516.684525563 -255883.940474005;-4e-05 -0.00040631202455906 339117.77786882 -253758.223625456;-2e-05 -0.000407352220181143 340705.483422869 -251622.488836743]  x2=[-0.00038 -0.000329528474463061 316167.909351575 -274630.341663344;-0.00036 -0.000330896720690628 317887.210439041 -272638.392204937;-0.00034 -0.000332251903682248 319593.961883749 -270635.679449638;-0.00032 -0.000333593969937617 321288.096306073 -268622.282461116;-0.0003 -0.000334922866474258 322969.546824489 -266598.280724838;-0.00028 -0.00033623854082961 324638.247058209 -264563.754144927;-0.00026 -0.000337540941063102 326294.131129805 -262518.783041007;-0.00024 -0.000338830015758204 327937.133667809 -260463.448145037;-0.00022 -0.000340105714024454 329567.189809294 -258397.83059812;-0.0002 -0.000341367985499468 331184.235202434 -256322.011947298;-0.00018 -0.000342616780350931 332788.206009047 -254236.074142338;-0.00016 -0.000343852049278559 334379.038907112 -252140.099532493;-0.00014 -0.00034507374351605 335956.671093269 -250034.170863251;-0.00012 -0.000346281814833009 337521.040285301 -247918.371273071;-0.0001 -0.000347476215536847 339072.084724592 -245792.784290097;-8e-05 -0.00034865689847467 340609.743178561 -243657.493828864;-6e-05 -0.000349823817035138 342133.954943088 -241512.584186983;-4e-05 -0.000350976925150304 343644.6598449 -239358.140041814;-2e-05 -0.000352116177297434 345141.798243956 -237194.246447123]  x3=[-0.00038 -3.05530268384323e-07 1574.64888181013 -1169.47388647692;-0.00036 -3.03535352930101e-07 1581.96577236795 -1159.55705644633;-0.00034 -3.01528454419881e-07 1589.22020962585 -1149.59444908862;-0.00032 -2.9950965208258e-07 1596.41190719105 -1139.58645771049;-0.0003 -2.97479025617057e-07 1603.54058114764 -1129.53347741029;-0.00028 -2.95436655188968e-07 1610.6059500678 -1119.43590506247;-0.00026 -2.93382621427601e-07 1617.60773502284 -1109.2941393019;-0.00024 -2.91317005422692e-07 1624.5456595943 -1099.10858050813;-0.00022 -2.89239888721224e-07 1631.41944988478 -1088.87963078957;-0.0002 -2.87151353324206e-07 1638.22883452882 -1078.60769396766;-0.00018 -2.85051481683442e-07 1644.97354470357 -1068.29317556085;-0.00016 -2.82940356698266e-07 1651.65331413941 -1057.93648276869;-0.00014 -2.8081806171228e-07 1658.2678791305 -1047.53802445566;-0.00012 -2.78684680510055e-07 1664.81697854513 -1037.0982111351;-0.0001 -2.76540297313828e-07 1671.30035383608 -1026.61745495296;-8e-05 -2.74384996780176e-07 1677.71774905077 -1016.09616967155;-6e-05 -2.72218863996673e-07 1684.06891084145 -1005.5347706532;-4e-05 -2.70041984478533e-07 1690.35358847511 -994.933674843854;-2e-05 -2.67854444165232e-07 1696.57153384346 -984.293300756623]  x4=[-0.00038 -6.12185239320934e-07 371.3787512776 -717.272178732514;-0.00036 -6.18085617328539e-07 375.878144937533 -714.924594240005;-0.00034 -6.23961594374304e-07 380.36269957191 -712.548785748662;-0.00032 -6.29812938484716e-07 384.832238138194 -710.144847051336;-0.0003 -6.3563941865873e-07 389.286584186654 -707.712873051412;-0.00028 -6.41440804876884e-07 393.725561867336 -705.252959759058;-0.00026 -6.47216868110384e-07 398.148995937001 -702.76520428744;-0.00024 -6.52967380330143e-07 402.556711766047 -700.249704848882;-0.00022 -6.58692114515787e-07 406.948535345401 -697.706560750997;-0.0002 -6.64390844664611e-07 411.324293293386 -695.135872392759;-0.00018 -6.70063345800507e-07 415.683812862572 -692.537741260542;-0.00016 -6.75709393982843e-07 420.026921946591 -689.912269924114;-0.00014 -6.81328766315305e-07 424.353449086932 -687.259562032589;-0.00012 -6.86921240954693e-07 428.663223479714 -684.579722310331;-0.0001 -6.92486597119687e-07 432.956074982421 -681.872856552825;-8e-05 -6.98024615099554e-07 437.231834120627 -679.139071622496;-6e-05 -7.03535076262825e-07 441.490332094683 -676.378475444491;-4e-05 -7.09017763065931e-07 445.731400786381 -673.591177002421;-2e-05 -7.14472459061784e-07 449.95487276559 -670.777286334056]  x5=0.000371346567279139  V1=[7.818e-10 4.235e+05 4.235e+05;314.2 314.2 314.2;1.708 0.8658 -0.705]  V2=[9.391e-10 4.188e+05 4.188e+05;314.2 314.2 314.2;1.235 0.8998 -0.671]  I1=[4.724e-12 1961 1961;314.2 314.2 314.2;-0.8175 0.9762 -0.5946]  I2=[5.7e-12 807.8 807.8;314.2 314.2 314.2;1.598 0.522 -1.049]  nHarmo=1  Measurements=None  Decoupling=off  VsMag0=0  VrMag0=0  VsAngle0=0  VrAngle0=0  IsMag0=0  IrMag0=0  IsAngle0=0  IrAngle0=0
      settings: SourceProductBaseCode=PS
  Line_69_b : spsDistributedParametersLineLib/Distributed Parameters Line  Phases=3  Length=70  Frequency=50  Resistance=[0.0298 0.1619]  Inductance=[1.0568e-03 3.9470e-03]  Capacitance=[11.0414e-09 7.1301e-09]  x1=[-0.00038 -0.000329528461531173 316167.909351575 -274630.341663344;-0.00036 -0.000330896707668672 317887.210439041 -272638.392204937;-0.00034 -0.000332251890570739 319593.961883749 -270635.679449638;-0.00032 -0.000333593956737073 321288.096306073 -268622.282461116;-0.0003 -0.000334922853185199 322969.546824489 -266598.280724838;-0.00028 -0.000336238527452561 324638.247058209 -264563.754144927;-0.00026 -0.000337540927598591 326294.131129805 -262518.783041007;-0.00024 -0.000338830002206763 327937.133667809 -260463.448145037;-0.00022 -0.000340105700386617 329567.189809294 -258397.83059812;-0.0002 -0.000341367971775775 331184.235202434 -256322.011947298;-0.00018 -0.000342616766541922 332788.206009047 -254236.074142338;-0.00016 -0.00034385203538478 334379.038907112 -252140.099532493;-0.00014 -0.000345073729538051 335956.671093269 -250034.170863251;-0.00012 -0.000346281800771339 337521.040285301 -247918.371273071;-0.0001 -0.000347476201392063 339072.084724592 -245792.784290097;-8e-05 -0.000348656884247331 340609.743178561 -243657.493828864;-6e-05 -0.000349823802725804 342133.954943088 -241512.584186983;-4e-05 -0.00035097691075954 343644.6598449 -239358.140041814;-2e-05 -0.000352116162825808 345141.798243956 -237194.246447123]  x2=[-0.00038 -0.000268754608279637 320559.859976877 -259085.927766452;-0.00036 -0.000270162036121011 322181.406580677 -257066.689883258;-0.00034 -0.00027155879842779 323790.234014208 -255037.303447317;-0.00032 -0.000272944840058191 325386.278763717 -252997.848575329;-0.0003 -0.000274320106293663 326969.477820092 -250948.405781481;-0.00028 -0.00027568454284105 328539.768681344 -248889.055974265;-0.00026 -0.000277038095834732 330097.089355078 -246819.880453286;-0.00024 -0.000278380711838757 331641.378360941 -244740.96090605;-0.00022 -0.000279712337848942 333172.574733048 -242652.379404741;-0.0002 -0.000281032921294973 334690.618022387 -240554.21840298;-0.00018 -0.000282342410042477 336195.448299209 -238446.560732572;-0.00016 -0.00028364075239508 337687.00615539 -236329.489600232;-0.00014 -0.000284927897096449 339165.232706782 -234203.088584303;-0.00012 -0.000286203793332316 340630.069595529 -232067.441631457;-0.0001 -0.000287468390732481 342081.458992382 -229922.633053378;-8e-05 -0.000288721639372804 343519.343598971 -227768.747523437;-6e-05 -0.000289963489777176 344943.666650073 -225605.870073347;-4e-05 -0.000291193892919469 346354.371915855 -223434.086089805;-2e-05 -0.000292412800225473 347751.403704087 -221253.481311125]  x3=[-0.00038 -2.63555567121397e-07 1662.23209254417 -1049.16655312505;-0.00036 -2.61291402545705e-07 1668.79134598867 -1038.70179993513;-0.00034 -2.59016922632844e-07 1675.28471840826 -1028.19604057668;-0.00032 -2.56732217175385e-07 1681.71195345571 -1017.64968979911;-0.0003 -2.54437376369588e-07 1688.07279739479 -1007.06316395429;-0.00028 -2.52132490811839e-07 1694.36699911027 -996.436880980115;-0.00026 -2.49817651495072e-07 1700.59431011785 -985.771260384055;-0.00024 -2.4749294980518e-07 1706.75448457395 -975.066723226546;-0.00022 -2.45158477517407e-07 1712.84727928542 -964.323692104386;-0.0002 -2.42814326792719e-07 1718.87245371918 -953.542591134048;-0.00018 -2.40460590174174e-07 1724.82977001165 -942.723845934938;-0.00016 -2.38097360583263e-07 1730.71899297818 -931.867883612593;-0.00014 -2.35724731316245e-07 1736.53989012233 -920.975132741816;-0.00012 -2.3334279604046e-07 1742.29223164505 -910.046023349761;-0.0001 -2.30951648790634e-07 1747.97579045375 -899.080986898952;-8e-05 -2.28551383965166e-07 1753.59034217125 -888.080456270253;-6e-05 -2.26142096322402e-07 1759.13566514467 -877.044865745778;-4e-05 -2.23723880976893e-07 1764.61154045416 -865.974650991745;-2e-05 -2.21296833395639e-07 1770.01775192153 -854.870249041277]  x4=[-0.00038 -4.96869478284107e-07 320.889568163653 -744.355774623379;-0.00036 -5.03115356453991e-07 325.560128569359 -742.32488633027;-0.00034 -5.09341372491074e-07 330.217836418638 -740.264692321711;-0.00032 -5.15547280602902e-07 334.862507833159 -738.175273930636;-0.0003 -5.21732835790851e-07 339.493959449247 -736.056713643705;-0.00028 -5.27897793859793e-07 344.112008425122 -733.90909509805;-0.00026 -5.34041911427738e-07 348.716472448119 -731.732503077975;-0.00024 -5.40164945935447e-07 353.307169741882 -729.527023511604;-0.00022 -5.46266655656001e-07 357.883919073543 -727.292743467496;-0.0002 -5.52346799704348e-07 362.446539760874 -725.0297511512;-0.00018 -5.58405138046812e-07 366.994851679423 -722.738135901779;-0.00016 -5.64441431510568e-07 371.528675269623 -720.417988188278;-0.00014 -5.70455441793087e-07 376.047831543883 -718.069399606156;-0.00012 -5.7644693147154e-07 380.55214209365 -715.69246287367;-0.0001 -5.82415664012174e-07 385.041429096458 -713.287271828212;-8e-05 -5.88361403779647e-07 389.515515322941 -710.853921422605;-6e-05 -5.94283916046336e-07 393.974224143836 -708.392507721357;-4e-05 -6.00182967001597e-07 398.417379536954 -705.903127896866;-2e-05 -6.06058323760998e-07 402.844806094128 -703.385880225586]  x5=0.000371346567279139  V1=[9.514e-10 4.188e+05 4.188e+05;314.2 314.2 314.2;1.248 0.8998 -0.671]  V2=[3.385e-10 4.122e+05 4.122e+05;314.2 314.2 314.2;1.899 0.9353 -0.6355]  I1=[9.51e-12 1966 1966;314.2 314.2 314.2;2.181 1.052 -0.5188]  I2=[1.088e-11 810.7 810.7;314.2 314.2 314.2;-0.4113 0.4513 -1.119]  nHarmo=1  Measurements=None  Decoupling=off  VsMag0=0  VrMag0=0  VsAngle0=0  VrAngle0=0  IsMag0=0  IrMag0=0  IsAngle0=0  IrAngle0=0
      settings: SourceProductBaseCode=PS
  Line_78_a : spsDistributedParametersLineLib/Distributed Parameters Line  Phases=3  Length=100  Frequency=50  Resistance=[0.0298 0.1619]  Inductance=[1.0568e-03 3.9470e-03]  Capacitance=[11.0414e-09 7.1301e-09]  x1=[-0.00054 -7.86116219991208e-05 302306.480951241 -277089.945200239;-0.00052 -8.27932942288857e-05 304041.509693409 -275185.040541629;-0.0005 -8.69716979211592e-05 305764.535397377 -273269.272048811;-0.00048 -9.11466681197183e-05 307475.49004104 -271342.715353045;-0.00046 -9.5318040003888e-05 309174.306078839 -269405.446511489;-0.00044 -9.94856488950491e-05 310860.916444425 -267457.542004202;-0.00042 -0.000103649330263138 312535.254553309 -265499.078731116;-0.0004 -0.000107808919733145 314197.254305489 -263530.13400901;-0.00038 -0.000111964253091599 315846.850088061 -261550.785568449;-0.00036 -0.000116115166293055 317483.976777808 -259561.11155072;-0.00034 -0.000120261495466566 319108.569743772 -257561.190504747;-0.00032 -0.000124403076922157 320720.564849803 -255551.101383989;-0.0003 -0.000128539747157283 322319.898457096 -253530.923543321;-0.00028 -0.000132671342863287 323906.507426698 -251500.736735906;-0.00026 -0.000136797700931844 325480.329122003 -249460.621110043;-0.00024 -0.000140918658461404 327041.301411226 -247410.657206004;-0.00022 -0.000145034052763618 328589.362669854 -245350.925952853;-0.0002 -0.000149143721369768 330124.451783079 -243281.508665254;-0.00018 -0.000153247502037174 331646.508148211 -241202.487040257;-0.00016 -0.0001573452327556 333155.471677071 -239113.943154076;-0.00014 -0.000161436751753656 334651.282798363 -237015.959458849;-0.00012 -0.000165521897505176 336133.882460024 -234908.618779378;-0.0001 -0.000169600508735601 337603.21213156 -232792.004309866;-8e-05 -0.000173672424428345 339059.21380635 -230666.199610628;-6e-05 -0.000177737483831147 340501.830003941 -228531.288604793;-4e-05 -0.000181795526462422 341931.003772316 -226387.355574991;-2e-05 -0.000185846392117596 343346.678690142 -224234.485160029]  x2=[-0.00054 1.48220438794773e-05 278378.632660918 -309253.440627953;-0.00052 1.17895679991099e-05 280316.221591206 -307498.243205379;-0.0005 8.75662668678494e-06 282242.744117044 -305730.906278685;-0.00048 5.72333967783213e-06 284158.124182621 -303951.499619306;-0.00046 2.68982672122875e-06 286062.286172011 -302160.09347517;-0.00044 -3.43792425127842e-07 287955.154912161 -300356.758567925;-0.00042 -3.37739799914818e-06 289836.655675854 -298541.566090144;-0.0004 -6.41087023927853e-06 291706.714184659 -296714.58770252;-0.00038 -9.44408938922899e-06 293565.256611871 -294875.89553103;-0.00036 -1.24769357027013e-05 295412.209585416 -293025.562164092;-0.00034 -1.55092894481159e-05 297247.500190753 -291163.660649701;-0.00032 -1.85410309133393e-05 299071.055973752 -289290.264492539;-0.0003 -2.15720404104096e-05 300882.804943553 -287405.447651079;-0.00028 -2.46021982802617e-05 302682.675575409 -285509.284534663;-0.00026 -2.76313848974514e-05 304470.596813508 -283601.850000564;-0.00024 -3.06594806748779e-05 306246.498073783 -281683.219351031;-0.00022 -3.36863660685047e-05 308010.309246691 -279753.468330316;-0.0002 -3.67119215820795e-05 309761.960699989 -277812.673121687;-0.00018 -3.97360277718511e-05 311501.383281476 -275860.910344414;-0.00016 -4.27585652512853e-05 313228.508321726 -273898.257050751;-0.00014 -4.57794146957777e-05 314943.267636801 -271924.790722888;-0.00012 -4.87984568473648e-05 316645.593530939 -269940.589269897;-0.0001 -5.1815572519432e-05 318335.418799229 -267945.731024654;-8e-05 -5.48306426014185e-05 320012.676730262 -265940.294740747;-6e-05 -5.78435480635203e-05 321677.301108767 -263924.359589366;-4e-05 -6.08541699613885e-05 323329.226218224 -261898.00515618;-2e-05 -6.38623894408257e-05 324968.386843458 -259861.311438191]  x3=[-0.00054 -1.37818042793668e-06 -99.8584639562027 -314.331095974709;-0.00052 -1.37793540670088e-06 -97.8815053079144 -314.952316438569;-0.0005 -1.37763598693462e-06 -95.9006824653965 -315.56110312426;-0.00048 -1.37728218045849e-06 -93.9160736281432 -316.157431997927;-0.00046 -1.37687400124017e-06 -91.9277571451131 -316.741279517527;-0.00044 -1.37641146539386e-06 -89.9358115116364 -317.31262263376;-0.00042 -1.37589459117969e-06 -87.940315366316 -317.871438790977;-0.0004 -1.37532339900296e-06 -85.941347487923 -318.417705928074;-0.00038 -1.37469791141338e-06 -83.9389867922862 -318.951402479359;-0.00036 -1.37401815310412e-06 -81.9333123291775 -319.472507375407;-0.00034 -1.37328415091086e-06 -79.9244032791903 -319.981000043888;-0.00032 -1.37249593381077e-06 -77.9123389506141 -320.476860410383;-0.0003 -1.3716535329213e-06 -75.8971987763035 -320.960068899172;-0.00028 -1.37075698149899e-06 -73.879062310542 -321.430606434014;-0.00026 -1.36980631493817e-06 -71.8580092259017 -321.888454438891;-0.00024 -1.36880157076952e-06 -69.8341193100977 -322.333594838747;-0.00022 -1.36774278865862e-06 -67.8074724628386 -322.766010060203;-0.0002 -1.36663001040437e-06 -65.7781486926716 -323.185683032246;-0.00018 -1.36546327993736e-06 -63.7462281138245 -323.592597186905;-0.00016 -1.36424264331811e-06 -61.7117909430425 -323.986736459907;-0.00014 -1.36296814873525e-06 -59.6749174964215 -324.368085291307;-0.00012 -1.36163984650366e-06 -57.6356881862376 -324.736628626107;-0.0001 -1.36025778906242e-06 -55.5941835177722 -325.092351914847;-8e-05 -1.35882203097281e-06 -53.5504840861341 -325.435241114181;-6e-05 -1.35733262891609e-06 -51.5046705730773 -325.76528268743;-4e-05 -1.35578964169131e-06 -49.4568237438164 -326.082463605118;-2e-05 -1.35419313021296e-06 -47.4070244438378 -326.386771345485]  x4=[-0.00054 1.42135215849248e-06 1862.00304861866 -1667.59919523511;-0.00052 1.41152115450041e-06 1872.44406007242 -1655.86704506055;-0.0005 1.40163442607007e-06 1882.81115064083 -1644.06952409035;-0.00048 1.39169236351258e-06 1893.10391104891 -1632.20709807044;-0.00046 1.38169535932353e-06 1903.32193495608 -1620.28023530908;-0.00044 1.37164380816754e-06 1913.46481897227 -1608.2894066584;-0.00042 1.36153810686263e-06 1923.53216267379 -1596.23508549577;-0.0004 1.35137865436459e-06 1933.52356861914 -1584.11774770516;-0.00038 1.34116585175121e-06 1943.43864236472 -1571.93787165832;-0.00036 1.33090010220644e-06 1953.27699248041 -1559.69593819589;-0.00034 1.3205818110045e-06 1963.03823056497 -1547.39243060845;-0.00032 1.31021138549386e-06 1972.72197126145 -1535.02783461741;-0.0003 1.29978923508117e-06 1982.32783227235 -1522.60263835585;-0.00028 1.28931577121507e-06 1991.85543437472 -1510.11733234923;-0.00026 1.27879140736998e-06 2001.30440143514 -1497.57240949607;-0.00024 1.26821655902978e-06 2010.67436042458 -1484.96836504844;-0.00022 1.25759164367135e-06 2019.96494143309 -1472.30569659243;-0.0002 1.24691708074818e-06 2029.17577768445 -1459.58490402851;-0.00018 1.23619329167372e-06 2038.30650555061 -1446.80648955179;-0.00016 1.22542069980481e-06 2047.35676456607 -1433.97095763219;-0.00014 1.21459973042493e-06 2056.3261974421 -1421.07881499454;-0.00012 1.20373081072742e-06 2065.21445008085 -1408.13057059854;-0.0001 1.19281436979862e-06 2074.02117158933 -1395.12673561873;-8e-05 1.18185083860092e-06 2082.74601429324 -1382.06782342423;-6e-05 1.17084064995577e-06 2091.38863375075 -1368.95434955854;-4e-05 1.15978423852656e-06 2099.94868876602 -1355.78683171916;-2e-05 1.14868204080148e-06 2108.42584140275 -1342.56578973714]  x5=0.000530495096113056  V1=[8.92e-10 4.101e+05 4.101e+05;314.2 314.2 314.2;-0.7547 0.8912 -0.6796]  V2=[4.527e-10 4.161e+05 4.161e+05;314.2 314.2 314.2;-0.9521 0.7952 -0.7756]  I1=[5.472e-12 329.9 329.9;314.2 314.2 314.2;0.6215 -0.2451 -1.816]  I2=[4.185e-12 2499 2499;314.2 314.2 314.2;-1.63 0.9027 -0.6681]  nHarmo=1  Measurements=None  Decoupling=off  VsMag0=0  VrMag0=0  VsAngle0=0  VrAngle0=0  IsMag0=0  IrMag0=0  IsAngle0=0  IrAngle0=0
      settings: SourceProductBaseCode=PS
  Line_78_b : spsDistributedParametersLineLib/Distributed Parameters Line  Phases=3  Length=10  Frequency=50  Resistance=[0.0298 0.1619]  Inductance=[1.0568e-03 3.9470e-03]  Capacitance=[11.0414e-09 7.1301e-09]  x1=[-6e-05 -5.78435478578096e-05 0 0;-4e-05 -6.08541698242436e-05 323329.226218224 -261898.00515618;-2e-05 -6.38623893722518e-05 324968.386843458 -259861.311438191]  x2=[-6e-05 -4.58192365546322e-05 0 0;-4e-05 -4.87198961278785e-05 321274.698353668 -265270.987804589;-2e-05 -5.16186323230476e-05 322935.09246916 -263247.136401205]  x3=[-6e-05 -1.33717889238232e-06 0 0;-4e-05 -1.334073695538e-06 -22.6247847025794 -328.35354104521;-2e-05 -1.33091583174847e-06 -20.5612455358813 -328.489214392254]  x4=[-6e-05 1.20862508947825e-06 0 0;-4e-05 1.19758032147816e-06 2095.55384429237 -1385.57459717307;-2e-05 1.18648827505756e-06 2104.21824449844 -1372.38058064693]  x5=5.30495096113055e-05  V1=[4.527e-10 4.161e+05 4.161e+05;314.2 314.2 314.2;-0.8021 0.8918 -0.679]  V2=[3.459e-10 4.166e+05 4.166e+05;314.2 314.2 314.2;-1.332 0.8824 -0.6884]  I1=[2.305e-11 329.2 329.2;314.2 314.2 314.2;1.554 -0.06674 -1.638]  I2=[1.894e-11 2512 2512;314.2 314.2 314.2;-2.04 0.9884 -0.5824]  nHarmo=1  Measurements=None  Decoupling=off  VsMag0=0  VrMag0=0  VsAngle0=0  VrAngle0=0  IsMag0=0  IrMag0=0  IsAngle0=0  IrAngle0=0
      settings: SourceProductBaseCode=PS
  Line_89_a : spsDistributedParametersLineLib/Distributed Parameters Line  Phases=3  Length=100  Frequency=50  Resistance=[0.0298 0.1619]  Inductance=[1.0568e-03 3.9470e-03]  Capacitance=[11.0414e-09 7.1301e-09]  x1=[-0.00054 2.40426038328311e-05 275822.474002518 -312264.756805445;-0.00052 2.11301884881824e-05 277779.033922328 -310525.560654946;-0.0005 1.82169389598729e-05 279724.627601512 -308774.105487018;-0.00048 1.53029702580057e-05 281659.178231364 -307010.460446111;-0.00046 1.23883974210755e-05 283582.609439137 -305234.695157911;-0.00044 9.47333551142755e-06 285494.845291061 -303446.879726593;-0.00042 6.55789961071451e-06 287395.810295337 -301647.084732047;-0.0004 3.64220481535376e-06 289285.429405124 -299835.381227098;-0.00038 7.26366231983364e-07 291163.628021494 -298011.840734699;-0.00036 -2.18950102708214e-06 293030.331996382 -296176.535245106;-0.00034 -5.1052818483961e-06 294885.467635511 -294329.537213037;-0.00032 -8.02086112192435e-06 296728.961701302 -292470.919554811;-0.0003 -1.09361237455894e-05 298560.741415767 -290600.755645472;-0.00028 -1.38509546298146e-05 300380.734463378 -288719.119315888;-0.00026 -1.67652387020677e-05 302188.868993927 -286826.08484984;-0.00024 -1.96788609114035e-05 303985.073625359 -284921.726981087;-0.00022 -2.25917062330062e-05 305769.277446589 -283006.120890417;-0.0002 -2.55036596727299e-05 307541.410020307 -281079.342202678;-0.00018 -2.8414606271639e-05 309301.401385753 -279141.466983794;-0.00016 -3.13244311105462e-05 311049.18206148 -277192.57173776;-0.00014 -3.42330193145491e-05 312784.683048101 -275232.733403624;-0.00012 -3.71402560575657e-05 314507.835831009 -273262.029352446;-0.0001 -4.00460265668676e-05 316218.572383082 -271280.53738425;-8e-05 -4.29502161276103e-05 317916.82516737 -269288.335724944;-6e-05 -4.58527100873629e-05 319602.527139761 -267285.50302324;-4e-05 -4.87533938606337e-05 321275.611751628 -265272.118347542;-2e-05 -5.1652152933394e-05 322936.012952455 -263248.26118283]  x2=[-0.00054 -0.000231569722429994 304441.989310742 -278441.264238236;-0.00052 -0.000233188054019842 306185.466433075 -276522.915199255;-0.0005 -0.000234797179744598 307916.855877466 -274593.649509064;-0.00048 -0.000236397036078735 309636.089291625 -272653.543331771;-0.00046 -0.000237987559862664 311343.098803161 -270702.673259444;-0.00044 -0.00023956868830523 313037.817022261 -268741.116309094;-0.00042 -0.000241140358986188 314720.177044352 -266768.949919631;-0.0004 -0.000242702509858673 316390.11245274 -264786.251948807;-0.00038 -0.000244255079251641 318047.557321235 -262793.100670142;-0.00036 -0.000245798005872313 319692.446216751 -260789.574769837;-0.00034 -0.000247331228808586 321324.714201893 -258775.753343663;-0.00032 -0.000248854687531445 322944.296837513 -256751.715893842;-0.0003 -0.000250368321897347 324551.130185264 -254717.542325908;-0.00028 -0.0002518720721506 326145.150810115 -252673.312945548;-0.00026 -0.000253365878925719 327726.295782863 -250619.108455439;-0.00024 -0.000254849683249769 329294.50268261 -248555.009952057;-0.00022 -0.000256323426544697 330849.709599234 -246481.098922477;-0.0002 -0.000257787050629642 332391.855135828 -244397.457241154;-0.00018 -0.00025924049772323 333920.878411127 -242304.167166695;-0.00016 -0.000260683710445858 335436.719061911 -240201.311338607;-0.00014 -0.00026211663182196 336939.317245386 -238088.972774039;-0.00012 -0.000263539205282253 338428.613641549 -235967.234864498;-0.0001 -0.000264951374665973 339904.549455528 -233836.181372566;-8e-05 -0.000266353084223091 341367.066419904 -231695.896428585;-6e-05 -0.000267744278616513 342816.106797012 -229546.46452734;-4e-05 -0.000269124902924267 344251.613381218 -227387.970524722;-2e-05 -0.000270494902641669 345673.529501182 -225220.499634378]  x3=[-0.00054 -1.79504755453719e-06 1915.2535545649 -1812.17451505855;-0.00052 -1.81018420594905e-06 1926.60190244914 -1800.10493046174;-0.0005 -1.825249394388e-06 1937.87419138914 -1787.96428080455;-0.00048 -1.84024252510619e-06 1949.06997637423 -1775.75304537904;-0.00046 -1.85516300620048e-06 1960.188815414 -1763.47170626387;-0.00044 -1.87001024863584e-06 1971.23026955572 -1751.12074830529;-0.00042 -1.88478366626855e-06 1982.19390290168 -1738.70065909796;-0.0004 -1.89948267586938e-06 1993.07928262642 -1726.21192896575;-0.00038 -1.91410669714661e-06 2003.88597899377 -1713.65505094232;-0.00036 -1.92865515276891e-06 2014.61356537388 -1701.03052075174;-0.00034 -1.94312746838816e-06 2025.26161826 -1688.33883678882;-0.00032 -1.95752307266213e-06 2035.82971728523 -1675.58050009953;-0.0003 -1.97184139727701e-06 2046.31744523912 -1662.75601436115;-0.00028 -1.98608187696985e-06 2056.72438808414 -1649.86588586241;-0.00026 -2.00024394955091e-06 2067.05013497198 -1636.91062348353;-0.00024 -2.01432705592581e-06 2077.29427825985 -1623.89073867607;-0.00022 -2.02833064011762e-06 2087.45641352652 -1610.80674544279;-0.0002 -2.04225414928881e-06 2097.53613958828 -1597.65916031734;-0.00018 -2.0560970337631e-06 2107.5330585148 -1584.44850234388;-0.00016 -2.06985874704709e-06 2117.44677564485 -1571.17529305655;-0.00014 -2.08353874585191e-06 2127.27689960185 -1557.84005645894;-0.00012 -2.09713649011464e-06 2137.02304230933 -1544.44331900335;-0.0001 -2.11065144301961e-06 2146.68481900627 -1530.98560957003;-8e-05 -2.12408307101962e-06 2156.26184826226 -1517.46745944632;-6e-05 -2.137430843857e-06 2165.7537519926 -1503.88940230562;-4e-05 -2.15069423458453e-06 2175.16015547318 -1490.2519741864;-2e-05 -2.16387271958627e-06 2184.48068735529 -1476.55571347095]  x4=[-0.00054 1.60079146061387e-06 -155.21259206971 -183.683013449754;-0.00052 1.60979092552815e-06 -154.055421487093 -184.654610784829;-0.0005 1.6187268386531e-06 -152.892169060222 -185.618918272049;-0.00048 1.62759884721416e-06 -151.72288071231 -186.575897842207;-0.00046 1.63640660095963e-06 -150.547602604858 -187.525511715386;-0.00044 1.64514975217447e-06 -149.366381135834 -188.467722402459;-0.00042 1.65382795569404e-06 -148.179262937839 -189.402492706559;-0.0004 1.66244086891772e-06 -146.986294876267 -190.329785724556;-0.00038 1.67098815182246e-06 -145.787524047454 -191.24956484851;-0.00036 1.67946946697615e-06 -144.58299777682 -192.161793767115;-0.00034 1.687884479551e-06 -143.372763616999 -193.066436467136;-0.00032 1.69623285733672e-06 -142.156869345965 -193.963457234828;-0.0003 1.70451427075364e-06 -140.93536296514 -194.852820657347;-0.00028 1.71272839286575e-06 -139.708292697505 -195.734491624148;-0.00026 1.72087489939358e-06 -138.475706985693 -196.60843532837;-0.00024 1.72895346872698e-06 -137.237654490078 -197.474617268214;-0.00022 1.73696378193788e-06 -135.994184086853 -198.333003248298;-0.0002 1.74490552279283e-06 -134.745344866098 -199.183559381015;-0.00018 1.7527783777655e-06 -133.49118612985 -200.026252087864;-0.00016 1.76058203604904e-06 -132.231757390146 -200.86104810078;-0.00014 1.76831618956841e-06 -130.967108367078 -201.687914463447;-0.00012 1.77598053299245e-06 -129.697288986823 -202.506818532596;-0.0001 1.78357476374602e-06 -128.422349379677 -203.317727979296;-8e-05 1.79109858202188e-06 -127.142339878071 -204.120610790232;-6e-05 1.79855169079258e-06 -125.857311014589 -204.915435268963;-4e-05 1.80593379582213e-06 -124.567313519971 -205.702170037182;-2e-05 1.81324460567769e-06 -123.272398321108 -206.480784035947]  x5=0.000530495096113056  V1=[5.499e-10 4.166e+05 4.166e+05;314.2 314.2 314.2;-1.286 0.7858 -0.785]  V2=[5.945e-10 4.126e+05 4.126e+05;314.2 314.2 314.2;-0.5426 0.8923 -0.6785]  I1=[4.251e-12 2637 2637;314.2 314.2 314.2;-0.8207 0.8753 -0.6955]  I2=[3.147e-12 240.5 240.5;314.2 314.2 314.2;2.253 -0.6397 -2.211]  nHarmo=1  Measurements=None  Decoupling=off  VsMag0=0  VrMag0=0  VsAngle0=0  VrAngle0=0  IsMag0=0  IrMag0=0  IsAngle0=0  IrAngle0=0
      settings: SourceProductBaseCode=PS
  Line_89_b : spsDistributedParametersLineLib/Distributed Parameters Line  Phases=3  Length=10  Frequency=50  Resistance=[0.0298 0.1619]  Inductance=[1.0568e-03 3.9470e-03]  Capacitance=[11.0414e-09 7.1301e-09]  x1=[-6e-05 -0.000267744278616513 0 0;-4e-05 -0.000269124902924267 344251.613381218 -227387.970524722;-2e-05 -0.000270494902641669 345673.529501182 -225220.499634378]  x2=[-6e-05 -0.000289688472317203 0 0;-4e-05 -0.000290914043084836 346349.120271208 -223429.067650337;-2e-05 -0.000292128129064172 347746.12063153 -221248.495967559]  x3=[-6e-05 -2.53305858885099e-06 0 0;-4e-05 -2.54420970704731e-06 2346.56677919426 -1260.74061470193;-2e-05 -2.55526038420077e-06 2354.44187474426 -1245.97191184872]  x4=[-6e-05 1.78972865861669e-06 0 0;-4e-05 1.79734318268201e-06 -123.74462031454 -207.368426480706;-2e-05 1.80488675071601e-06 -122.439252025644 -208.141838489235]  x5=5.30495096113055e-05  V1=[5.916e-10 4.126e+05 4.126e+05;314.2 314.2 314.2;-0.4212 0.9888 -0.582]  V2=[6.139e-10 4.122e+05 4.122e+05;314.2 314.2 314.2;-0.1116 0.9997 -0.5711]  I1=[1.499e-11 2664 2664;314.2 314.2 314.2;1.83 1.08 -0.4912]  I2=[2.162e-11 241.5 241.5;314.2 314.2 314.2;2.618 -0.5367 -2.107]  nHarmo=1  Measurements=None  Decoupling=off  VsMag0=0  VrMag0=0  VsAngle0=0  VrAngle0=0  IsMag0=0  IrMag0=0  IsAngle0=0  IrAngle0=0
      settings: SourceProductBaseCode=PS
  Ln_45 : spsThreePhaseVIMeasurementLib/Three-Phase V-I Measurement  VoltageMeasurement=phase-to-ground  SetLabelV=on  LabelV=Vabc_Ln_45  Vpu=off  VpuLL=off  CurrentMeasurement=yes  SetLabelI=on  LabelI=Iabc_Ln_45  Ipu=off  Pbase=100e6  Vbase=500e3  OutputType=Complex  PhasorSimulation=off  PSBequivalent=0
  Ln_46 : spsThreePhaseVIMeasurementLib/Three-Phase V-I Measurement  VoltageMeasurement=phase-to-ground  SetLabelV=on  LabelV=Vabc_Ln_46  Vpu=off  VpuLL=off  CurrentMeasurement=yes  SetLabelI=on  LabelI=Iabc_Ln_46  Ipu=off  Pbase=100e6  Vbase=500e3  OutputType=Complex  PhasorSimulation=off  PSBequivalent=0
  Ln_54 : spsThreePhaseVIMeasurementLib/Three-Phase V-I Measurement  VoltageMeasurement=phase-to-ground  SetLabelV=on  LabelV=Vabc_Ln_54  Vpu=off  VpuLL=off  CurrentMeasurement=yes  SetLabelI=on  LabelI=Iabc_Ln_54  Ipu=off  Pbase=100e6  Vbase=500e3  OutputType=Complex  PhasorSimulation=off  PSBequivalent=0
  Ln_57 : spsThreePhaseVIMeasurementLib/Three-Phase V-I Measurement  VoltageMeasurement=phase-to-ground  SetLabelV=on  LabelV=Vabc_Ln_57  Vpu=off  VpuLL=off  CurrentMeasurement=yes  SetLabelI=on  LabelI=Iabc_Ln_57  Ipu=off  Pbase=100e6  Vbase=500e3  OutputType=Complex  PhasorSimulation=off  PSBequivalent=0
  Ln_64 : spsThreePhaseVIMeasurementLib/Three-Phase V-I Measurement  VoltageMeasurement=phase-to-ground  SetLabelV=on  LabelV=Vabc_Ln_64  Vpu=off  VpuLL=off  CurrentMeasurement=yes  SetLabelI=on  LabelI=Iabc_Ln_64  Ipu=off  Pbase=100e6  Vbase=500e3  OutputType=Complex  PhasorSimulation=off  PSBequivalent=0
  Ln_69 : spsThreePhaseVIMeasurementLib/Three-Phase V-I Measurement  VoltageMeasurement=phase-to-ground  SetLabelV=on  LabelV=Vabc_Ln_69  Vpu=off  VpuLL=off  CurrentMeasurement=yes  SetLabelI=on  LabelI=Iabc_Ln_69  Ipu=off  Pbase=100e6  Vbase=500e3  OutputType=Complex  PhasorSimulation=off  PSBequivalent=0
  Ln_75 : spsThreePhaseVIMeasurementLib/Three-Phase V-I Measurement  VoltageMeasurement=phase-to-ground  SetLabelV=on  LabelV=Vabc_Ln_75  Vpu=off  VpuLL=off  CurrentMeasurement=yes  SetLabelI=on  LabelI=Iabc_Ln_75  Ipu=off  Pbase=100e6  Vbase=500e3  OutputType=Complex  PhasorSimulation=off  PSBequivalent=0
  Ln_78 : spsThreePhaseVIMeasurementLib/Three-Phase V-I Measurement  VoltageMeasurement=phase-to-ground  SetLabelV=on  LabelV=Vabc_Ln_78  Vpu=off  VpuLL=off  CurrentMeasurement=yes  SetLabelI=on  LabelI=Iabc_Ln_78  Ipu=off  Pbase=100e6  Vbase=500e3  OutputType=Complex  PhasorSimulation=off  PSBequivalent=0
  Ln_87 : spsThreePhaseVIMeasurementLib/Three-Phase V-I Measurement  VoltageMeasurement=phase-to-ground  SetLabelV=on  LabelV=Vabc_Ln_87  Vpu=off  VpuLL=off  CurrentMeasurement=yes  SetLabelI=on  LabelI=Iabc_Ln_87  Ipu=off  Pbase=100e6  Vbase=500e3  OutputType=Complex  PhasorSimulation=off  PSBequivalent=0
  Ln_89 : spsThreePhaseVIMeasurementLib/Three-Phase V-I Measurement  VoltageMeasurement=phase-to-ground  SetLabelV=on  LabelV=Vabc_Ln_89  Vpu=off  VpuLL=off  CurrentMeasurement=yes  SetLabelI=on  LabelI=Iabc_Ln_89  Ipu=off  Pbase=100e6  Vbase=500e3  OutputType=Complex  PhasorSimulation=off  PSBequivalent=0
  Ln_96 : spsThreePhaseVIMeasurementLib/Three-Phase V-I Measurement  VoltageMeasurement=phase-to-ground  SetLabelV=on  LabelV=Vabc_Ln_96  Vpu=off  VpuLL=off  CurrentMeasurement=yes  SetLabelI=on  LabelI=Iabc_Ln_96  Ipu=off  Pbase=100e6  Vbase=500e3  OutputType=Complex  PhasorSimulation=off  PSBequivalent=0
  Ln_98 : spsThreePhaseVIMeasurementLib/Three-Phase V-I Measurement  VoltageMeasurement=phase-to-ground  SetLabelV=on  LabelV=Vabc_Ln_98  Vpu=off  VpuLL=off  CurrentMeasurement=yes  SetLabelI=on  LabelI=Iabc_Ln_98  Ipu=off  Pbase=100e6  Vbase=500e3  OutputType=Complex  PhasorSimulation=off  PSBequivalent=0
  "Load A 1020 MW, 320 MVAR" : spsThreePhaseParallelRLCLoadLib/Three-Phase Parallel RLC Load  LConnTagsString=A|B|C  Configuration=Y (grounded)  NominalVoltage=(400000)*1.04156  Vabc=[1e3 1e3 1e3]  Vabcp=[1e3 1e3 1e3]  NominalFrequency=50  UnbalancedPower=off  ActivePower=1020000000  InductivePower=320000000  CapacitivePower=0  Pabc=[10e3 9e3 11e3]  QLabc=[100 90 110]  QCabc=[100 90 110]  Pabcp=[10e3 9e3 11e3]  QLabcp=[100 90 110]  QCabcp=[100 90 110]  Measurements=None  LoadType=constant PQ
  "Load B 850 MW, 250 MVAR" : spsThreePhaseParallelRLCLoadLib/Three-Phase Parallel RLC Load  LConnTagsString=A|B|C  Configuration=Y (grounded)  NominalVoltage=(400000)*1.05047  Vabc=[1e3 1e3 1e3]  Vabcp=[1e3 1e3 1e3]  NominalFrequency=50  UnbalancedPower=off  ActivePower=850000000  InductivePower=280000000  CapacitivePower=0  Pabc=[10e3 9e3 11e3]  QLabc=[100 90 110]  QCabc=[100 90 110]  Pabcp=[10e3 9e3 11e3]  QLabcp=[100 90 110]  QCabcp=[100 90 110]  Measurements=None  LoadType=constant PQ
  "Load C 360 MW, 120 MVAR" : spsThreePhaseParallelRLCLoadLib/Three-Phase Parallel RLC Load  LConnTagsString=A|B|C  Configuration=Y (grounded)  NominalVoltage=(400000)*1.05886  Vabc=[1e3 1e3 1e3]  Vabcp=[1e3 1e3 1e3]  NominalFrequency=50  UnbalancedPower=off  ActivePower=360000000  InductivePower=120000000  CapacitivePower=0  Pabc=[10e3 9e3 11e3]  QLabc=[100 90 110]  QCabc=[100 90 110]  Pabcp=[10e3 9e3 11e3]  QLabcp=[100 90 110]  QCabcp=[100 90 110]  Measurements=None  LoadType=constant PQ
  Load Flow Bus : spsLoadFlowBusLib/Load Flow Bus  LConnTagsString=a  Phases=single  Connectors=on one side  ID=BUS_1  Vbase=24e3  Vref=1  Vangle=0  VLF=1  VLFb=1  VLFc=1  angleLF=0  angleLFb=0  angleLFc=0
      settings: SourceProductBaseCode=PS
  Load Flow Bus1 : spsLoadFlowBusLib/Load Flow Bus  LConnTagsString=a  Phases=single  Connectors=on one side  ID=BUS_4  Vbase=400e3  Vref=1  Vangle=0  VLF=1.038  VLFb=1  VLFc=1  angleLF=25.46  angleLFb=0  angleLFc=0
      settings: SourceProductBaseCode=PS
  Load Flow Bus2 : spsLoadFlowBusLib/Load Flow Bus  LConnTagsString=a  Phases=single  Connectors=on one side  ID=BUS_5  Vbase=400e3  Vref=1  Vangle=0  VLF=1.05  VLFb=1  VLFc=1  angleLF=20.03  angleLFb=0  angleLFc=0
      settings: SourceProductBaseCode=PS
  Load Flow Bus3 : spsLoadFlowBusLib/Load Flow Bus  LConnTagsString=a  Phases=single  Connectors=on one side  ID=BUS_2  Vbase=26e3  Vref=1  Vangle=0  VLF=1  VLFb=1  VLFc=1  angleLF=4.046  angleLFb=0  angleLFc=0
      settings: SourceProductBaseCode=PS
  Load Flow Bus4 : spsLoadFlowBusLib/Load Flow Bus  LConnTagsString=a  Phases=single  Connectors=on one side  ID=BUS_7  Vbase=400e3  Vref=1  Vangle=0  VLF=1.025  VLFb=1  VLFc=1  angleLF=27.21  angleLFb=0  angleLFc=0
      settings: SourceProductBaseCode=PS
  Load Flow Bus5 : spsLoadFlowBusLib/Load Flow Bus  LConnTagsString=a  Phases=single  Connectors=on one side  ID=BUS_8  Vbase=400e3  Vref=1  Vangle=0  VLF=1.042  VLFb=1  VLFc=1  angleLF=21.17  angleLFb=0  angleLFc=0
      settings: SourceProductBaseCode=PS
  Load Flow Bus6 : spsLoadFlowBusLib/Load Flow Bus  LConnTagsString=a  Phases=single  Connectors=on one side  ID=BUS_9  Vbase=400e3  Vref=1  Vangle=0  VLF=1.03  VLFb=1  VLFc=1  angleLF=27.89  angleLFb=0  angleLFc=0
      settings: SourceProductBaseCode=PS
  Load Flow Bus7 : spsLoadFlowBusLib/Load Flow Bus  LConnTagsString=a  Phases=single  Connectors=on one side  ID=BUS_3  Vbase=26e3  Vref=1  Vangle=0  VLF=1  VLFb=1  VLFc=1  angleLF=4.557  angleLFb=0  angleLFc=0
      settings: SourceProductBaseCode=PS
  Load Flow Bus8 : spsLoadFlowBusLib/Load Flow Bus  LConnTagsString=a  Phases=single  Connectors=on one side  ID=BUS_6  Vbase=400e3  Vref=1  Vangle=0  VLF=1.059  VLFb=1  VLFc=1  angleLF=23.91  angleLFb=0  angleLFc=0
      settings: SourceProductBaseCode=PS
  Power Balance : Subsystem  Commented=on
  Rotor Angle Deviations : Scope  Commented=on  NumInputPorts=2
  Scope : Scope  NumInputPorts=2
  Scope1 : Scope  Commented=on  NumInputPorts=3
  Scope2 : Scope  NumInputPorts=2
  Scope3 : Scope
  Shunt Compensation 200 MVAr : spsThreePhaseParallelRLCLoadLib/Three-Phase Parallel RLC Load  LConnTagsString=A|B|C  Configuration=Y (grounded)  NominalVoltage=(400000)*0.905282  Vabc=[1e3 1e3 1e3]  Vabcp=[1e3 1e3 1e3]  NominalFrequency=50  UnbalancedPower=off  ActivePower=0  InductivePower=0  CapacitivePower=200000000  Pabc=[10e3 9e3 11e3]  QLabc=[100 90 110]  QCabc=[100 90 110]  Pabcp=[10e3 9e3 11e3]  QLabcp=[100 90 110]  QCabcp=[100 90 110]  Measurements=None  LoadType=constant Z
  Shunt Compensation 350 MVAr : spsThreePhaseParallelRLCLoadLib/Three-Phase Parallel RLC Load  LConnTagsString=A|B|C  Configuration=Y (grounded)  NominalVoltage=(400000)*0.905282  Vabc=[1e3 1e3 1e3]  Vabcp=[1e3 1e3 1e3]  NominalFrequency=50  UnbalancedPower=off  ActivePower=0  InductivePower=0  CapacitivePower=350000000  Pabc=[10e3 9e3 11e3]  QLabc=[100 90 110]  QCabc=[100 90 110]  Pabcp=[10e3 9e3 11e3]  QLabcp=[100 90 110]  QCabcp=[100 90 110]  Measurements=None  LoadType=constant Z
  Shunt Compensation 400 MVAr : spsThreePhaseParallelRLCLoadLib/Three-Phase Parallel RLC Load  LConnTagsString=A|B|C  Configuration=Y (grounded)  NominalVoltage=(400000)*0.905282  Vabc=[1e3 1e3 1e3]  Vabcp=[1e3 1e3 1e3]  NominalFrequency=50  UnbalancedPower=off  ActivePower=0  InductivePower=0  CapacitivePower=400000000  Pabc=[10e3 9e3 11e3]  QLabc=[100 90 110]  QCabc=[100 90 110]  Pabcp=[10e3 9e3 11e3]  QLabcp=[100 90 110]  QCabcp=[100 90 110]  Measurements=None  LoadType=constant Z
  Snb_G1 : spsThreePhaseSeriesRLCLoadLib/Three-Phase Series RLC Load  LConnTagsString=A|B|C  Configuration=Y (grounded)  NominalVoltage=26e3  Vabc=[1e3 1e3 1e3]  Vabcp=[1e3 1e3 1e3]  NominalFrequency=50  UnbalancedPower=off  ActivePower=1000000  InductivePower=0  CapacitivePower=10000000  Pabc=[10e3 9e3 11e3]  QLabc=[100 90 110]  QCabc=[100 90 110]  Pabcp=[10e3 9e3 11e3]  QLabcp=[100 90 110]  QCabcp=[100 90 110]  Measurements=None  LoadType=constant Z
  Snb_G2 : spsThreePhaseSeriesRLCLoadLib/Three-Phase Series RLC Load  LConnTagsString=A|B|C  Configuration=Y (grounded)  NominalVoltage=26e3  Vabc=[1e3 1e3 1e3]  Vabcp=[1e3 1e3 1e3]  NominalFrequency=50  UnbalancedPower=off  ActivePower=1000000  InductivePower=0  CapacitivePower=10000000  Pabc=[10e3 9e3 11e3]  QLabc=[100 90 110]  QCabc=[100 90 110]  Pabcp=[10e3 9e3 11e3]  QLabcp=[100 90 110]  QCabcp=[100 90 110]  Measurements=None  LoadType=constant Z
  Snb_G3 : spsThreePhaseSeriesRLCLoadLib/Three-Phase Series RLC Load  LConnTagsString=A|B|C  Configuration=Y (grounded)  NominalVoltage=26e3  Vabc=[1e3 1e3 1e3]  Vabcp=[1e3 1e3 1e3]  NominalFrequency=50  UnbalancedPower=off  ActivePower=1000000  InductivePower=0  CapacitivePower=10000000  Pabc=[10e3 9e3 11e3]  QLabc=[100 90 110]  QCabc=[100 90 110]  Pabcp=[10e3 9e3 11e3]  QLabcp=[100 90 110]  QCabcp=[100 90 110]  Measurements=None  LoadType=constant Z
  Source 1 776.5MVA,24kV,50Hz1 : spsThreePhaseSourceLib/Three-Phase Source  InternalConnection=Yg  VoltagePhases=off  Voltage=(24000)*1.02752  PhaseAngle=35.9818  Voltage_phases=[25e3 25e3 25e3]/sqrt(3)  PhaseAngles_phases=[0 -120 +120]  Frequency=50  NonIdealSource=on  SpecifyImpedance=on  Resistance=0.8929  Inductance=16.58e-3  ShortCircuitLevel=776.5e6  BaseVoltage=24e3  XRratio=7  BusType=swing  Pref=1020000000  Qref=0  Prefabc=[10e3, 10e3, 10e3]  Qrefabc=[0, 0, 0]  Qmin=-Inf  Qmax=Inf
  Source 2 1200MVA,26kV,50Hz : spsThreePhaseSourceLib/Three-Phase Source  InternalConnection=Yg  VoltagePhases=off  Voltage=(26000)*1.31746  PhaseAngle=45.2983  Voltage_phases=[25e3 25e3 25e3]/sqrt(3)  PhaseAngles_phases=[0 -120 +120]  Frequency=50  NonIdealSource=on  SpecifyImpedance=on  Resistance=0.8929  Inductance=16.58e-3  ShortCircuitLevel=1200e6  BaseVoltage=26e3  XRratio=7  BusType=PV  Pref=1020000000  Qref=0  Prefabc=[10e3, 10e3, 10e3]  Qrefabc=[0, 0, 0]  Qmin=-Inf  Qmax=Inf
  Source 3 960MVA,26kV,50Hz1 : spsThreePhaseSourceLib/Three-Phase Source  InternalConnection=Yg  VoltagePhases=off  Voltage=(26000)*1.27823  PhaseAngle=46.709  Voltage_phases=[25e3 25e3 25e3]/sqrt(3)  PhaseAngles_phases=[0 -120 +120]  Frequency=50  NonIdealSource=on  SpecifyImpedance=on  Resistance=0.8929  Inductance=16.58e-3  ShortCircuitLevel=960e6  BaseVoltage=26e3  XRratio=7  BusType=PV  Pref=800000000  Qref=0  Prefabc=[10e3, 10e3, 10e3]  Qrefabc=[0, 0, 0]  Qmin=-Inf  Qmax=Inf
  Subsystem_1 : Subsystem
  Subsystem_2 : Subsystem
  Subsystem_3 : Subsystem
  Subsystem_4 : Subsystem
  Subsystem_5 : Subsystem
  Subsystem_6 : Subsystem
  Subsystem_7 : Subsystem
  Subsystem_75 : Subsystem
  Subsystem_78 : Subsystem
  Subsystem_8 : Subsystem
  Subsystem_87 : Subsystem
  Subsystem_9 : Subsystem
  Subtract : Sum  Commented=on  Inputs=+-
  Subtract1 : Sum  Commented=on  Inputs=+-
  Three-Phase Breaker10 : spsThreePhaseBreakerLib/Three-Phase Breaker  InitialState=closed  SwitchA=on  SwitchB=on  SwitchC=on  SwitchTimes=[(0.5+(10/50)) ]  External=off  BreakerResistance=0.01  SnubberResistance=inf  SnubberCapacitance=inf  Measurements=None
  Three-Phase Breaker{4..9,12..13} (8 alike) : spsThreePhaseBreakerLib/Three-Phase Breaker  InitialState=closed  SwitchA=on  SwitchB=on  SwitchC=on  SwitchTimes=[500 501]  External=off  BreakerResistance=0.01  SnubberResistance=10e6  SnubberCapacitance=inf  Measurements=None
  Three-Phase Fault1 : spsThreePhaseFaultLib/Three-Phase Fault  InitialStates=0  FaultA=on  FaultB=on  FaultC=on  GroundFault=off  SwitchTimes=[0.5 0.5+(10/50)]  External=off  SwitchStatus=NaN  FaultResistance=0.001  GroundResistance=0.01  SnubberResistance=inf  SnubberCapacitance=inf  Measurements=None
  Xmer_1 800 MVA 24 kV /400 kV : spsThreePhaseTransformerTwoWindingsLib/Three-Phase Transformer (Two Windings)  Winding1Connection=Delta (D1)  Winding2Connection=Yg  CoreType=Three single-phase transformers  SetSaturation=off  Hysteresis=off  DataFile='hysteresis'  SetInitialFlux=off  Measurements=None  UNITS=pu  NominalPower=[ 800e6 50 ]  Winding1="[ 24e3 1e-6  0]"  Winding2=[ 400e3 1e-6 0.15]  Rm=500  Lm=500  L0=0.5  Saturation="[ 0,0  ;  0.005,1.2  ;  1.0,1.4 ]"  InitialFluxes=[ 0.8 , -0.8 , 0.7 ]  BreakLoop=off  DiscreteSolver=Trapezoidal iterative  DataType=off  TransfoNumber=0
  Xmer_2 1250 MVA 26 kV / 400 kV : spsThreePhaseTransformerTwoWindingsLib/Three-Phase Transformer (Two Windings)  Winding1Connection=Delta (D1)  Winding2Connection=Yg  CoreType=Three single-phase transformers  SetSaturation=off  Hysteresis=off  DataFile='hysteresis'  SetInitialFlux=off  Measurements=None  UNITS=pu  NominalPower=[ 1250e6 50 ]  Winding1="[ 26e3 1e-6  0]"  Winding2=[ 400e3 1e-6 0.15]  Rm=500  Lm=500  L0=0.5  Saturation="[ 0,0  ;  0.005,1.2  ;  1.0,1.4 ]"  InitialFluxes=[ 0.8 , -0.8 , 0.7 ]  BreakLoop=off  DiscreteSolver=Trapezoidal iterative  DataType=off  TransfoNumber=0
  Xmer_3 1000 MVA 26 kV / 400 kV : spsThreePhaseTransformerTwoWindingsLib/Three-Phase Transformer (Two Windings)  Winding1Connection=Delta (D1)  Winding2Connection=Yg  CoreType=Three single-phase transformers  SetSaturation=off  Hysteresis=off  DataFile='hysteresis'  SetInitialFlux=off  Measurements=None  UNITS=pu  NominalPower=[1000e6 50 ]  Winding1="[ 26e3 1e-6  0]"  Winding2=[ 400e3 1e-6 0.15]  Rm=500  Lm=500  L0=0.5  Saturation="[ 0,0  ;  0.005,1.2  ;  1.0,1.4 ]"  InitialFluxes=[ 0.8 , -0.8 , 0.7 ]  BreakLoop=off  DiscreteSolver=Trapezoidal iterative  DataType=off  TransfoNumber=0
  powergui : spspowerguiLib/powergui  Priority=2  SimulationMode=Discrete  SampleTime=20e-6  frequency=60  Iterations=50  frequencyindice=50  Pbase=100e6  ErrMax=0.0001  UnitsV=kV  UnitsW=MW  buscounter=0  FunctionMessages=off  echomessages=off  EnableUseOfTLC=off  CurrentSourceSwitches=off  DisableSnubberDevices=off  DisableRonSwitches=off  DisableVfSwitches=off  DisplayEquations=off  AutomaticDiscreteSolvers=off  SolverType=Tustin  Interpol=off  ExternalGateDelay=off  methode=off  Ts=100  x0status=blocks  SPID=on  SwTol=0  HookPort=off  NonlinearTolerance=1e-4  nMaxIteration=100  ContinueOnMaxIteration=off  RestoreLinks=warning  ResistiveCurrentMeasurement=off  Frange=logspace(0,3,50)  Ylog=off  Xlog=off  ShowGrid=off  save=off  variable=ZData  structure=0  ZoomFFT=on  StartTime=0.0  cycles=2  DisplayStyle=off  fundamental=60  FreqAxis=off  MaxFrequency=1000  frequencyindicesteady=1  RmsSteady=1  display=off
  tag scope: PSS=global
  wires:
  Subtract1/1 -> Gain/1
  Subtract/1 -> Gain1/1
  Gain/1 -> Rotor Angle Deviations/1
  Gain1/1 -> Rotor Angle Deviations/2
  Gain2/1 -> Scope1/1
  Gain3/1 -> Scope1/2
  Gain4/1 -> Scope1/3
  From/1 -> Gain3/1, Subtract1/1
  From2/1 -> Gain4/1, Subtract/1
  From1/1 -> Gain2/1, Subtract1/2, Subtract/2
  Constant/1 -> [PSS]
  [Vabc_Ln_78] -> Demux/1
  [Iabc_Ln_78] -> Demux1/1
  Demux/1 -> Scope/1
  Demux1/1 -> Scope/2
  [Vabc_Ln_75] -> Subsystem_75/1(In1)
  [Iabc_Ln_75] -> Subsystem_75/2(In2)
  [Iabc_Ln_78] -> Subsystem_78/2(In2)
  [Vabc_Ln_78] -> Scope3/1, Subsystem_78/1(In1)
  [Iabc_Ln_87] -> Subsystem_87/2(In2)
  [Vabc_Ln_87] -> Subsystem_87/1(In1)
  [Vabc_Ln_57] -> Subsystem_1/1(In1)
  [Iabc_Ln_57] -> Subsystem_1/2(In2)
  [Vabc_Ln_54] -> Subsystem_2/1(In1)
  [Iabc_Ln_54] -> Subsystem_2/2(In2)
  [Vabc_Ln_45] -> Subsystem_3/1(In1)
  [Iabc_Ln_45] -> Subsystem_3/2(In2)
  [Vabc_Ln_46] -> Subsystem_4/1(In1)
  [Iabc_Ln_46] -> Subsystem_4/2(In2)
  [Vabc_Ln_64] -> Subsystem_5/1(In1)
  [Iabc_Ln_64] -> Subsystem_5/2(In2)
  [Iabc_Ln_69] -> Subsystem_6/2(In2)
  [Vabc_Ln_69] -> Subsystem_6/1(In1)
  [Iabc_Ln_96] -> Subsystem_7/2(In2)
  [Vabc_Ln_96] -> Subsystem_7/1(In1)
  [Vabc_Ln_89] -> Subsystem_8/1(In1)
  [Iabc_Ln_89] -> Subsystem_8/2(In2)
  [Vabc_Ln_98] -> Subsystem_9/1(In1)
  [Iabc_Ln_98] -> Subsystem_9/2(In2)
  [Vabc_Ln_75] -> Demux2/1
  Demux2/1 -> Scope2/1
  [Iabc_Ln_75] -> Demux3/1
  Demux3/1 -> Scope2/2
  connections:
  B2/RConn2 -- Snb_G2/LConn2 -- Xmer_2 1250 MVA 26 kV / 400 kV/LConn2
  B2/RConn3 -- Snb_G2/LConn3 -- Xmer_2 1250 MVA 26 kV / 400 kV/LConn3
  B2/RConn1 -- Snb_G2/LConn1 -- Load Flow Bus3/LConn1 -- Xmer_2 1250 MVA 26 kV / 400 kV/LConn1
  Xmer_3 1000 MVA 26 kV / 400 kV/LConn3 -- Snb_G3/LConn3 -- B3/RConn3
  Xmer_3 1000 MVA 26 kV / 400 kV/LConn2 -- B3/RConn2 -- Snb_G3/LConn2
  Xmer_3 1000 MVA 26 kV / 400 kV/LConn1 -- B3/RConn1 -- Load Flow Bus7/LConn1 -- Snb_G3/LConn1
  B7/LConn2 -- Xmer_2 1250 MVA 26 kV / 400 kV/RConn2
  B7/LConn3 -- Xmer_2 1250 MVA 26 kV / 400 kV/RConn3
  Source 2 1200MVA,26kV,50Hz/RConn1 -- B2/LConn1
  Source 2 1200MVA,26kV,50Hz/RConn2 -- B2/LConn2
  Source 2 1200MVA,26kV,50Hz/RConn3 -- B2/LConn3
  B7/LConn1 -- Xmer_2 1250 MVA 26 kV / 400 kV/RConn1
  Line_78_b/LConn1 -- Line_78_a/RConn1
  Line_78_b/LConn2 -- Line_78_a/RConn2
  Line_78_b/LConn3 -- Line_78_a/RConn3
  B9/LConn2 -- Xmer_3 1000 MVA 26 kV / 400 kV/RConn2
  B9/LConn1 -- Xmer_3 1000 MVA 26 kV / 400 kV/RConn1
  B9/LConn3 -- Xmer_3 1000 MVA 26 kV / 400 kV/RConn3
  B_78/LConn1 -- Ln_78/RConn1
  B_78/LConn2 -- Ln_78/RConn2
  B_78/LConn3 -- Ln_78/RConn3
  B_78/RConn1 -- Line_78_a/LConn1
  B_78/RConn2 -- Line_78_a/LConn2
  B_78/RConn3 -- Line_78_a/LConn3
  Line_78_b/RConn1 -- B_87/RConn1
  Line_78_b/RConn2 -- B_87/RConn2
  Line_78_b/RConn3 -- B_87/RConn3
  Ln_87/RConn1 -- B_87/LConn1
  Ln_87/RConn2 -- B_87/LConn2
  Ln_87/RConn3 -- B_87/LConn3
  Ln_78/LConn1 -- Ln_75/LConn1 -- Load Flow Bus4/LConn1 -- B7/RConn1
  Ln_78/LConn2 -- Ln_75/LConn2 -- B7/RConn2
  Ln_78/LConn3 -- Ln_75/LConn3 -- B7/RConn3
  Line_89_b/LConn1 -- Line_89_a/RConn1
  Three-Phase Breaker4/RConn2 -- Line_89_a/LConn2
  Line_89_b/LConn2 -- Line_89_a/RConn2
  Three-Phase Breaker4/RConn1 -- Line_89_a/LConn1
  Line_89_b/RConn1 -- Three-Phase Breaker5/RConn1
  Line_89_b/LConn3 -- Line_89_a/RConn3
  Three-Phase Breaker4/LConn1 -- Ln_89/RConn1
  Ln_98/RConn1 -- Three-Phase Breaker5/LConn1
  Three-Phase Breaker4/LConn2 -- Ln_89/RConn2
  Three-Phase Breaker4/LConn3 -- Ln_89/RConn3
  Line_89_b/RConn3 -- Three-Phase Breaker5/RConn3
  Ln_98/RConn2 -- Three-Phase Breaker5/LConn2
  Line_89_b/RConn2 -- Three-Phase Breaker5/RConn2
  Three-Phase Breaker4/RConn3 -- Line_89_a/LConn3
  Ln_98/RConn3 -- Three-Phase Breaker5/LConn3
  Ln_87/LConn1 -- B8/LConn1 -- Load Flow Bus5/LConn1 -- Shunt Compensation 400 MVAr/LConn1 -- Ln_89/LConn1
  Ln_87/LConn2 -- Shunt Compensation 400 MVAr/LConn2 -- Ln_89/LConn2 -- B8/LConn2
  Ln_87/LConn3 -- Shunt Compensation 400 MVAr/LConn3 -- B8/LConn3 -- Ln_89/LConn3
  Ln_98/LConn1 -- B9/RConn1 -- Load Flow Bus6/LConn1 -- Ln_96/LConn1
  Ln_98/LConn2 -- B9/RConn2 -- Ln_96/LConn2
  Ln_98/LConn3 -- Ln_96/LConn3 -- B9/RConn3
  B8/RConn1 -- "Load A 1020 MW, 320 MVAR"/LConn1
  B8/RConn2 -- "Load A 1020 MW, 320 MVAR"/LConn2
  B8/RConn3 -- "Load A 1020 MW, 320 MVAR"/LConn3
  B6/RConn3 -- "Load C 360 MW, 120 MVAR"/LConn3
  B6/RConn2 -- "Load C 360 MW, 120 MVAR"/LConn2
  B6/RConn1 -- "Load C 360 MW, 120 MVAR"/LConn1
  B5/RConn1 -- "Load B 850 MW, 250 MVAR"/LConn1
  B5/RConn2 -- "Load B 850 MW, 250 MVAR"/LConn2
  B5/RConn3 -- "Load B 850 MW, 250 MVAR"/LConn3
  Line_69_b/LConn1 -- Line_69_a/RConn1
  Three-Phase Breaker6/RConn2 -- Line_69_a/LConn2
  Line_69_b/LConn2 -- Line_69_a/RConn2
  Three-Phase Breaker6/RConn1 -- Line_69_a/LConn1
  Line_69_b/RConn1 -- Three-Phase Breaker7/RConn1
  Line_69_b/LConn3 -- Line_69_a/RConn3
  Three-Phase Breaker6/LConn1 -- Ln_69/RConn1
  Ln_96/RConn1 -- Three-Phase Breaker7/LConn1
  Three-Phase Breaker6/LConn2 -- Ln_69/RConn2
  Three-Phase Breaker6/LConn3 -- Ln_69/RConn3
  Line_69_b/RConn3 -- Three-Phase Breaker7/RConn3
  Ln_96/RConn2 -- Three-Phase Breaker7/LConn2
  Line_69_b/RConn2 -- Three-Phase Breaker7/RConn2
  Three-Phase Breaker6/RConn3 -- Line_69_a/LConn3
  Ln_96/RConn3 -- Three-Phase Breaker7/LConn3
  Ln_64/RConn3 -- Three-Phase Breaker9/LConn3
  Three-Phase Breaker8/RConn3 -- Line_46_a/LConn3
  Line_46_b/RConn2 -- Three-Phase Breaker9/RConn2
  Ln_64/RConn2 -- Three-Phase Breaker9/LConn2
  Three-Phase Breaker8/LConn2 -- Ln_46/RConn2
  Ln_64/RConn1 -- Three-Phase Breaker9/LConn1
  Line_46_b/LConn2 -- Line_46_a/RConn2
  Line_46_b/RConn3 -- Three-Phase Breaker9/RConn3
  Line_46_b/RConn1 -- Three-Phase Breaker9/RConn1
  Line_46_b/LConn3 -- Line_46_a/RConn3
  Three-Phase Breaker8/RConn2 -- Line_46_a/LConn2
  Three-Phase Breaker8/RConn1 -- Line_46_a/LConn1
  Three-Phase Breaker8/LConn1 -- Ln_46/RConn1
  Line_46_b/LConn1 -- Line_46_a/RConn1
  Three-Phase Breaker8/LConn3 -- Ln_46/RConn3
  Ln_69/LConn1 -- Shunt Compensation 200 MVAr/LConn1 -- B6/LConn1 -- Ln_64/LConn1 -- Load Flow Bus8/LConn1
  Ln_69/LConn2 -- Shunt Compensation 200 MVAr/LConn2 -- B6/LConn2 -- Ln_64/LConn2
  Ln_69/LConn3 -- B6/LConn3 -- Shunt Compensation 200 MVAr/LConn3 -- Ln_64/LConn3
  Ln_57/LConn1 -- B5/LConn1 -- Ln_54/LConn1 -- Shunt Compensation 350 MVAr/LConn1 -- Load Flow Bus2/LConn1
  Ln_57/LConn2 -- Shunt Compensation 350 MVAr/LConn2 -- B5/LConn2 -- Ln_54/LConn2
  Ln_57/LConn3 -- Shunt Compensation 350 MVAr/LConn3 -- B5/LConn3 -- Ln_54/LConn3
  Three-Phase Breaker12/LConn3 -- Ln_45/RConn3
  Line_45_b/LConn1 -- Line_45_a/RConn1
  Three-Phase Breaker12/RConn1 -- Line_45_a/LConn1
  Three-Phase Breaker12/LConn1 -- Ln_45/RConn1
  Line_45_b/LConn3 -- Line_45_a/RConn3
  Line_45_b/RConn1 -- Three-Phase Breaker13/RConn1
  Line_45_b/LConn2 -- Line_45_a/RConn2
  Ln_54/RConn1 -- Three-Phase Breaker13/LConn1
  Ln_54/RConn2 -- Three-Phase Breaker13/LConn2
  Line_45_b/RConn2 -- Three-Phase Breaker13/RConn2
  Three-Phase Breaker12/RConn3 -- Line_45_a/LConn3
  Ln_54/RConn3 -- Three-Phase Breaker13/LConn3
  Ln_75/RConn3 -- B_75/LConn3
  Three-Phase Breaker10/RConn3 -- Line_57_a/LConn3
  Line_57_b/RConn2 -- B_75/RConn2
  Ln_75/RConn2 -- B_75/LConn2
  Three-Phase Breaker12/LConn2 -- Ln_45/RConn2
  Line_45_b/RConn3 -- Three-Phase Breaker13/RConn3
  Three-Phase Breaker10/LConn2 -- Ln_57/RConn2
  Ln_75/RConn1 -- B_75/LConn1
  Three-Phase Breaker10/LConn1 -- Ln_57/RConn1
  Line_57_b/LConn2 -- Three-Phase Fault1/LConn2 -- Line_57_a/RConn2
  Line_57_b/RConn3 -- B_75/RConn3
  Line_57_b/RConn1 -- B_75/RConn1
  Line_57_b/LConn3 -- Three-Phase Fault1/LConn3 -- Line_57_a/RConn3
  Three-Phase Breaker10/RConn2 -- Line_57_a/LConn2
  Three-Phase Breaker10/RConn1 -- Line_57_a/LConn1
  Line_57_b/LConn1 -- Three-Phase Fault1/LConn1 -- Line_57_a/RConn1
  Three-Phase Breaker10/LConn3 -- Ln_57/RConn3
  Three-Phase Breaker12/RConn2 -- Line_45_a/LConn2
  Xmer_1 800 MVA 24 kV /400 kV/RConn1 -- B4/LConn1
  Xmer_1 800 MVA 24 kV /400 kV/RConn2 -- B4/LConn2
  Xmer_1 800 MVA 24 kV /400 kV/RConn3 -- B4/LConn3
  B1/RConn1 -- Load Flow Bus/LConn1 -- Snb_G1/LConn1 -- Xmer_1 800 MVA 24 kV /400 kV/LConn1
  B1/RConn2 -- Snb_G1/LConn2 -- Xmer_1 800 MVA 24 kV /400 kV/LConn2
  B1/RConn3 -- Snb_G1/LConn3 -- Xmer_1 800 MVA 24 kV /400 kV/LConn3
  Ln_45/LConn1 -- Load Flow Bus1/LConn1 -- B4/RConn1 -- Ln_46/LConn1
  Ln_45/LConn2 -- Ln_46/LConn2 -- B4/RConn2
  Ln_45/LConn3 -- Ln_46/LConn3 -- B4/RConn3
  Source 3 960MVA,26kV,50Hz1/RConn1 -- B3/LConn1
  Source 3 960MVA,26kV,50Hz1/RConn2 -- B3/LConn2
  Source 3 960MVA,26kV,50Hz1/RConn3 -- B3/LConn3
  Source 1 776.5MVA,24kV,50Hz1/RConn1 -- B1/LConn1
  Source 1 776.5MVA,24kV,50Hz1/RConn2 -- B1/LConn2
  Source 1 776.5MVA,24kV,50Hz1/RConn3 -- B1/LConn3
